simulink model "Pitoni_0"  (R2023a)
settings: Solver=VariableStepAuto  StartTime=0.0  StopTime=10  RelTol=1e-3
(part 1 of 2)
settings Model: Creator=Stefano  LastModifiedBy=hp
settings SolverCC: AlgebraicLoopSolver=TrustRegion
settings DebuggingCC: UnconnectedInputMsg=warning  UnconnectedOutputMsg=warning  UnconnectedLineMsg=warning
settings ModelReferenceCC: EnableRefExpFcnMdlSchedulingChecks=on
settings SFSimCC: CustomCodeUndefinedFunction=UseInterfaceOnly
settings RTWCC: DLArmComputeVersion=19.05

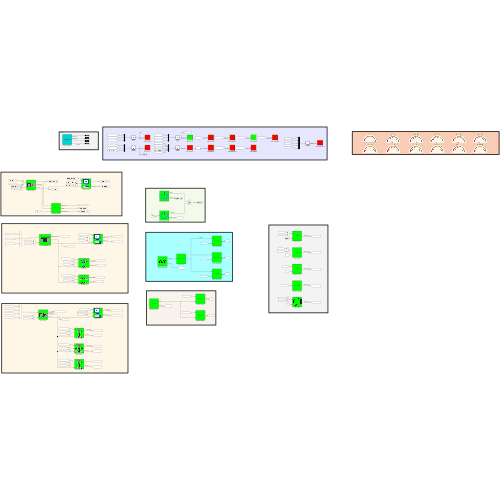
[thumbnail: Simulink's stored preview of the top-level diagram]
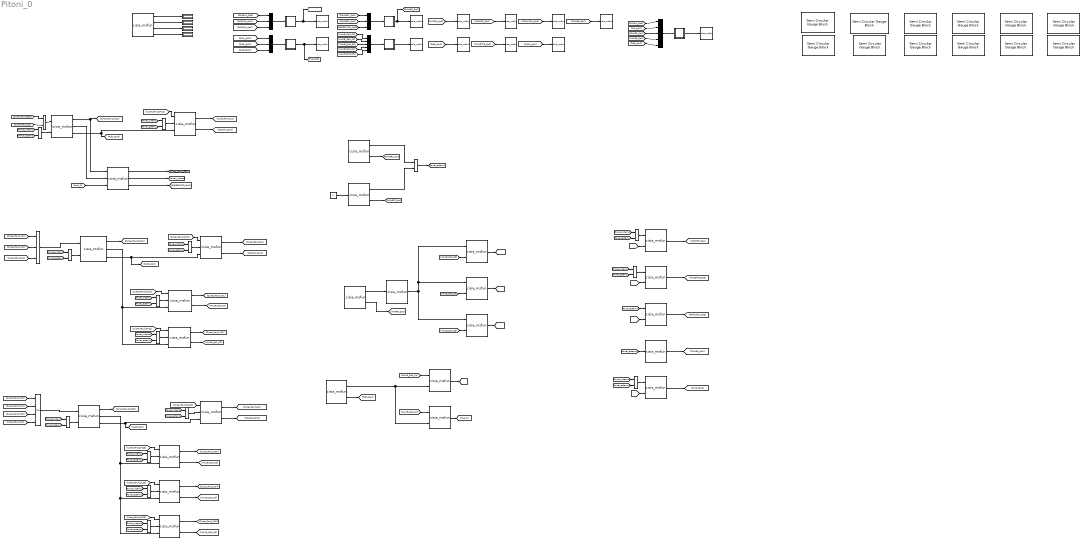
== system Pitoni_0 ==
  note: MASTER
  CISIA_MASTER (0) : M-S-Function  FunctionName=cisia_msfun  Parameters=Parameter1, Parameter2, Parameter3, resources, Parameter4, Parameter5, Parameter6, Parameter7, Parameter8, Parameter9,Parameter11  mask(S-function:msfcn_unit_delay){Parameter1='CISIA_MASTER', Parameter2=1, Parameter3='SistemiIoT', resources=off, Parameter4=on, Parameter5=off, Parameter6=off, Parameter7=off, Parameter8=0.001, Parameter9=off, Parameter11=on}
      mask prompts: Parameter1 "entity name"; Parameter2 "sampling time"; Parameter3 "project"; resources "Save status at each major hit"; Parameter4 "Show Operative Levels with colors"; Parameter5 "Load Entities from file"; Parameter6 "Load Start from Mask"; Parameter7 "Real Time"; Parameter8 "Real Time Hit (sec)"; Parameter9 "Skip saving"; Parameter11 "Show unconnected"
      mask help: This is a level-2 MATLAB file S-function which demonstrates CISIA entity
      mask Display: disp('MASTER BLOCK')
  CarWash_01 (491) : M-S-Function  FunctionName=cisia_msfun  Parameters=Parameter1, Parameter2, Parameter3, resources, Parameter10, codeupdate, step_received, step_computed, dynamic_computed, step_sended, id_entity, id_project, id_type, name_type, color  mask(S-function:msfcn_unit_delay){Parameter1='CarWash_01', Parameter2=1, Parameter3='', resources=|, Parameter10=off, codeupdate=off, step_received=|, step_computed=, dynamic_computed=, step_sended=CARWASH_QoS=Operative_Level;, id_entity=491, id_project=6, id_type=114, name_type=CarWash, color=#FFFFFF}
      mask resources=|
      | *** INPUT RESOURCES ***
      | NUM_INPUTS 2
      | POWER1 (1)
      | WATER1 (1)
      |
      | *** STATE VARIABLES ***
      | NUM_VARIABLES 3
      | Operative_Level(NUMERIC)(1)(1)
      | Power_Fault(NUMERIC)(1)(0)
      | Water_Fault(NUMERIC)(1)(0)
      |
      | *** OUTPUT RESOURCES ***
      | NUM_OUTPUTS 1
      | CARWASH_QoS (1)
      mask step_received=|
      | Power_Fault=1-POWER1;
      | Water_Fault=1-WATER1;
      |
      | Operative_Level=min(1-Power_Fault,1-Water_Fault);
      mask prompts: Parameter1 "entity name"; Parameter2 "sampling time"; Parameter3 "project"; resources "input resources and state variables"; Parameter10 "Bring state variables to output"; codeupdate "update code from mask"
      mask help: This is a level-2 MATLAB file S-function which demonstrates CISIA entity
      mask DialogControl Container1 Prompt: All parameters
      mask Display: disp('CarWash');port_label('input',1,'\color{yellow}\spadesuit','texmode','on');port_label('input',2,'\color{yellow}\spadesuit','texmode','on')
  Constant2 : Constant
  Display{18..21} (4 alike) : Display
  Fuel_Tank_01 (494) : M-S-Function  FunctionName=cisia_msfun  Parameters=Parameter1, Parameter2, Parameter3, resources, Parameter10, codeupdate, step_received, step_computed, dynamic_computed, step_sended, id_entity, id_project, id_type, name_type, color  mask(S-function:msfcn_unit_delay){Parameter1='Fuel_Tank_01', Parameter2=1, Parameter3='', resources=|, Parameter10=off, codeupdate=off, step_received=Operative_Level = 1-Mechanical_Fault, step_computed=, dynamic_computed=, step_sended=FUEL=Operative_Level;, id_entity=494, id_project=6, id_type=116, name_type=Fuel_Tank, color=#FFFFFF}
      mask resources=|
      | *** INPUT RESOURCES ***
      | NUM_INPUTS 0
      |
      | *** STATE VARIABLES ***
      | NUM_VARIABLES 2
      | Operative_Level(NUMERIC)(1)(1)
      | Mechanical_Fault(NUMERIC)(1)(0)
      |
      | *** OUTPUT RESOURCES ***
      | NUM_OUTPUTS 2
      | FUEL (1)
      | FUEL_QoS (1)
      mask prompts: Parameter1 "entity name"; Parameter2 "sampling time"; Parameter3 "project"; resources "input resources and state variables"; Parameter10 "Bring state variables to output"; codeupdate "update code from mask"
      mask help: This is a level-2 MATLAB file S-function which demonstrates CISIA entity
      mask DialogControl Container1 Prompt: All parameters
      mask Display: disp('Fuel_Tank')
  Fuel_pipe_01 (492) : M-S-Function  FunctionName=cisia_msfun  Parameters=Parameter1, Parameter2, Parameter3, resources, Parameter10, codeupdate, step_received, step_computed, dynamic_computed, step_sended, id_entity, id_project, id_type, name_type, color  mask(S-function:msfcn_unit_delay){Parameter1='Fuel_pipe_01', Parameter2=1, Parameter3='', resources=|, Parameter10=off, codeupdate=off, step_received=|, step_computed=, dynamic_computed=, step_sended=FUEL=1-Fuel_Fault;, id_entity=492, id_project=6, id_type=115, name_type=Fuel_Pipe, color=#FFFFFF}
      mask resources=|
      | *** INPUT RESOURCES ***
      | NUM_INPUTS 2
      | VALVE_QoS (1)
      | FUEL (1)
      |
      | *** STATE VARIABLES ***
      | NUM_VARIABLES 3
      | Operative_Level(NUMERIC)(1)(1)
      | Mechanical_Fault(NUMERIC)(1)(0)
      | Fuel_Fault(NUMERIC)(1)(0)
      |
      | *** OUTPUT RESOURCES ***
      | NUM_OUTPUTS 1
      | FUEL (1)
      mask step_received=|
      | Fuel_Fault=max([1-FUEL Mechanical_Fault 1-VALVE_QoS]);
      |
      | Operative_Level=1-Mechanical_Fault;
      mask prompts: Parameter1 "entity name"; Parameter2 "sampling time"; Parameter3 "project"; resources "input resources and state variables"; Parameter10 "Bring state variables to output"; codeupdate "update code from mask"
      mask help: This is a level-2 MATLAB file S-function which demonstrates CISIA entity
      mask DialogControl Container1 Prompt: All parameters
      mask Display: disp('Fuel_Pipe');port_label('input',1,'\color{yellow}\spadesuit','texmode','on')
  Fuel_pipe_02 (493) : M-S-Function  FunctionName=cisia_msfun  Parameters=Parameter1, Parameter2, Parameter3, resources, Parameter10, codeupdate, step_received, step_computed, dynamic_computed, step_sended, id_entity, id_project, id_type, name_type, color  mask(S-function:msfcn_unit_delay){Parameter1='Fuel_pipe_02', Parameter2=1, Parameter3='', resources=|, Parameter10=off, codeupdate=off, step_received=|, step_computed=, dynamic_computed=, step_sended=FUEL=1-Fuel_Fault;, id_entity=493, id_project=6, id_type=115, name_type=Fuel_Pipe, color=#FFFFFF}
      mask resources=|
      | *** INPUT RESOURCES ***
      | NUM_INPUTS 2
      | VALVE_QoS (1)
      | FUEL (1)
      |
      | *** STATE VARIABLES ***
      | NUM_VARIABLES 3
      | Operative_Level(NUMERIC)(1)(1)
      | Mechanical_Fault(NUMERIC)(1)(0)
      | Fuel_Fault(NUMERIC)(1)(0)
      |
      | *** OUTPUT RESOURCES ***
      | NUM_OUTPUTS 1
      | FUEL (1)
      mask step_received=|
      | Fuel_Fault=max([1-FUEL Mechanical_Fault 1-VALVE_QoS]);
      |
      | Operative_Level=1-Mechanical_Fault;
      mask prompts: Parameter1 "entity name"; Parameter2 "sampling time"; Parameter3 "project"; resources "input resources and state variables"; Parameter10 "Bring state variables to output"; codeupdate "update code from mask"
      mask help: This is a level-2 MATLAB file S-function which demonstrates CISIA entity
      mask DialogControl Container1 Prompt: All parameters
      mask Display: disp('Fuel_Pipe');port_label('input',1,'\color{yellow}\spadesuit','texmode','on')
  Generator_01 (495) : M-S-Function  FunctionName=cisia_msfun  Parameters=Parameter1, Parameter2, Parameter3, resources, Parameter10, codeupdate, step_received, step_computed, dynamic_computed, step_sended, id_entity, id_project, id_type, name_type, color  mask(S-function:msfcn_unit_delay){Parameter1='Generator_01', Parameter2=1, Parameter3='', resources=|, Parameter10=off, codeupdate=off, step_received=|, step_computed=, dynamic_computed=, step_sended=|, id_entity=495, id_project=6, id_type=117, name_type=Generator, color=#FFFFFF}
      mask resources=|
      | *** INPUT RESOURCES ***
      | NUM_INPUTS 3
      | CYBER_FAULT (10)
      | TELECONTROL (1)
      | FUEL (1)
      |
      | *** STATE VARIABLES ***
      | NUM_VARIABLES 14
      | Operative_Level(NUMERIC)(1)(1)
      | Dos_attack(NUMERIC)(1)(0)
      | MITM_attack(NUMERIC)(1)(0)
      | Virus_Attack(NUMERIC)(1)(0)
      | Port_Scan_Attack(NUMERIC)(1)(0)
      | Cyber_Fault(NUMERIC_ARRAY)(10)(0  0  0  0  0  0  0  0  0  0)
      | BGP_hijacking(NUMERIC)(1)(0)
      | Mechanical_Fault(NUMERIC)(1)(0)
      | BotNet_Attack(NUMERIC)(1)(0)
      | Data_Corruption(NUMERIC)(1)(0)
      | SW_Change(NUMERIC)(1)(0)
      | Config_Change(NUMERIC)(1)(0)
      | Port_Saturation(NUMERIC)(1)(0)
      | Control_Fault(NUMERIC)(1)(0)
      |
      | *** OUTPUT RESOURCES ***
      | NUM_OUTPUTS 3
      | CYBER_FAULT (10)
      | POWER1 (1)
      | GENERATOR_QoS (1)
      mask step_received=|
      | Cyber_Fault=max(CYBER_FAULT, transpose([Dos_attack MITM_attack Virus_Attack Port_Scan_Attack  BGP_hijacking BotNet_Attack Data_Corruption SW_Change Config_Change Port_Saturation]));
      |
      | Control_Fault=max([1-TELECONTROL Mechanical_Fault Dos_attack min(0.5,max(Cyber_Fault))]);
      |
      | Operative_Level=min([1-max(Cyber_Fault) 1-Mechanical_Fault FUEL]);
      mask step_sended=|
      | POWER1 = Operative_Level
      | GENERATOR_QoS = Operative_Level
      | CYBER_FAULT=Cyber_Fault.*transpose([0 0 0.5 0.2 0 0 0 0 0 0]);
      mask prompts: Parameter1 "entity name"; Parameter2 "sampling time"; Parameter3 "project"; resources "input resources and state variables"; Parameter10 "Bring state variables to output"; codeupdate "update code from mask"
      mask help: This is a level-2 MATLAB file S-function which demonstrates CISIA entity
      mask DialogControl Container1 Prompt: All parameters
      mask Display: disp('Generator');port_label('input',3,'\color{yellow}\spadesuit','texmode','on')
  Half Gauge{1..12} (12 alike) : SemiCircularGaugeBlock  ScaleMax=1
  Market_01 (517) : M-S-Function  FunctionName=cisia_msfun  Parameters=Parameter1, Parameter2, Parameter3, resources, Parameter10, codeupdate, step_received, step_computed, dynamic_computed, step_sended, id_entity, id_project, id_type, name_type, color  mask(S-function:msfcn_unit_delay){Parameter1='Market_01', Parameter2=1, Parameter3='', resources=|, Parameter10=off, codeupdate=off, step_received=|, step_computed=, dynamic_computed=, step_sended=MARKET_QoS=Operative_Level;, id_entity=517, id_project=6, id_type=128, name_type=Market, color=#FFFFFF}
      mask resources=|
      | *** INPUT RESOURCES ***
      | NUM_INPUTS 2
      | POWER1 (1)
      | WATER1 (1)
      |
      | *** STATE VARIABLES ***
      | NUM_VARIABLES 3
      | Operative_Level(NUMERIC)(1)(1)
      | Power_Fault(NUMERIC)(1)(0)
      | Water_Fault(NUMERIC)(1)(0)
      |
      | *** OUTPUT RESOURCES ***
      | NUM_OUTPUTS 1
      | MARKET_QoS (1)
      mask step_received=|
      | Power_Fault=1-POWER1;
      | Water_Fault=1-WATER1;
      |
      | Operative_Level=min(1-Power_Fault,1-Water_Fault);
      mask prompts: Parameter1 "entity name"; Parameter2 "sampling time"; Parameter3 "project"; resources "input resources and state variables"; Parameter10 "Bring state variables to output"; codeupdate "update code from mask"
      mask help: This is a level-2 MATLAB file S-function which demonstrates CISIA entity
      mask DialogControl Container1 Prompt: All parameters
      mask Display: disp('Market');port_label('input',1,'\color{yellow}\spadesuit','texmode','on');port_label('input',2,'\color{yellow}\spadesuit','texmode','on')
  MinMax : MinMax  Function=max  Inputs=4
  MinMax1 : MinMax  Function=max  Inputs=3
  MinMax{2..17} (16 alike) : MinMax  Function=max  Inputs=2
  Mux : Mux  Inputs=3
  Mux1 : Mux  Inputs=3
  Mux2 : Mux  Inputs=3
  Mux4 : Mux  Inputs=5
  Mux6 : Mux  Inputs=5
  PLC_01 (501) : M-S-Function  FunctionName=cisia_msfun  Parameters=Parameter1, Parameter2, Parameter3, resources, Parameter10, codeupdate, step_received, step_computed, dynamic_computed, step_sended, id_entity, id_project, id_type, name_type, color  mask(S-function:msfcn_unit_delay){Parameter1='PLC_01', Parameter2=1, Parameter3='', resources=|, Parameter10=off, codeupdate=off, step_received=|, step_computed=, dynamic_computed=, step_sended=|, id_entity=501, id_project=6, id_type=123, name_type=PLC, color=#FFFFFF}
      mask resources=|
      | *** INPUT RESOURCES ***
      | NUM_INPUTS 2
      | CYBER_FAULT (10)
      | POWER1 (1)
      |
      | *** STATE VARIABLES ***
      | NUM_VARIABLES 14
      | Operative_Level(NUMERIC)(1)(1)
      | Dos_attack(NUMERIC)(1)(0)
      | MITM_attack(NUMERIC)(1)(0)
      | Virus_Attack(NUMERIC)(1)(0)
      | Port_Scan_Attack(NUMERIC)(1)(0)
      | Cyber_Fault(NUMERIC_ARRAY)(10)(0  0  0  0  0  0  0  0  0  0)
      | BGP_hijacking(NUMERIC)(1)(0)
      | Mechanical_Fault(NUMERIC)(1)(0)
      | BotNet_Attack(NUMERIC)(1)(0)
      | Data_Corruption(NUMERIC)(1)(0)
      | SW_Change(NUMERIC)(1)(0)
      | Config_Change(NUMERIC)(1)(0)
      | Port_Saturation(NUMERIC)(1)(0)
      | Control_Fault(NUMERIC)(1)(0)
      |
      | *** OUTPUT RESOURCES ***
      | NUM_OUTPUTS 3
      | CYBER_FAULT (10)
      | TELECONTROL (1)
      | PLC_QoS (1)
      mask step_received=|
      | Cyber_Fault=max(CYBER_FAULT, transpose([Dos_attack MITM_attack Virus_Attack Port_Scan_Attack  BGP_hijacking BotNet_Attack Data_Corruption SW_Change Config_Change Port_Saturation]));
      |
      |
      | Control_Fault=max([Mechanical_Fault 1-POWER1 Dos_attack min(0.5,max(Cyber_Fault))]);
      |
      |
      |
      | Operative_Level=min([1-max(Cyber_Fault) 1-Mechanical_Fault 1-Control_Fault]);
      mask step_sended=|
      | CYBER_FAULT=Cyber_Fault.*transpose([0 0 0.5 0.2 0 0 0 0 0 0]);
      |
      | TELECONTROL=1-Control_Fault;
      | PLC_QoS=Operative_Level;
      mask prompts: Parameter1 "entity name"; Parameter2 "sampling time"; Parameter3 "project"; resources "input resources and state variables"; Parameter10 "Bring state variables to output"; codeupdate "update code from mask"
      mask help: This is a level-2 MATLAB file S-function which demonstrates CISIA entity
      mask DialogControl Container1 Prompt: All parameters
      mask Display: image('Icons/PLC.png');port_label('input',1,'\color{yellow}\spadesuit','texmode','on');port_label('input',2,'\color{yellow}\spadesuit','texmode','on')
  PLC_02 (506) : M-S-Function  FunctionName=cisia_msfun  Parameters=Parameter1, Parameter2, Parameter3, resources, Parameter10, codeupdate, step_received, step_computed, dynamic_computed, step_sended, id_entity, id_project, id_type, name_type, color  mask(S-function:msfcn_unit_delay){Parameter1='PLC_02', Parameter2=1, Parameter3='', resources=|, Parameter10=off, codeupdate=off, step_received=|, step_computed=, dynamic_computed=, step_sended=|, id_entity=506, id_project=6, id_type=123, name_type=PLC, color=#FFFFFF}
      mask resources=|
      | *** INPUT RESOURCES ***
      | NUM_INPUTS 2
      | CYBER_FAULT (10)
      | POWER1 (1)
      |
      | *** STATE VARIABLES ***
      | NUM_VARIABLES 14
      | Operative_Level(NUMERIC)(1)(1)
      | Dos_attack(NUMERIC)(1)(0)
      | MITM_attack(NUMERIC)(1)(0)
      | Virus_Attack(NUMERIC)(1)(0)
      | Port_Scan_Attack(NUMERIC)(1)(0)
      | Cyber_Fault(NUMERIC_ARRAY)(10)(0  0  0  0  0  0  0  0  0  0)
      | BGP_hijacking(NUMERIC)(1)(0)
      | Mechanical_Fault(NUMERIC)(1)(0)
      | BotNet_Attack(NUMERIC)(1)(0)
      | Data_Corruption(NUMERIC)(1)(0)
      | SW_Change(NUMERIC)(1)(0)
      | Config_Change(NUMERIC)(1)(0)
      | Port_Saturation(NUMERIC)(1)(0)
      | Control_Fault(NUMERIC)(1)(0)
      |
      | *** OUTPUT RESOURCES ***
      | NUM_OUTPUTS 3
      | CYBER_FAULT (10)
      | TELECONTROL (1)
      | PLC_QoS (1)
      mask step_received=|
      | Cyber_Fault=max(CYBER_FAULT, transpose([Dos_attack MITM_attack Virus_Attack Port_Scan_Attack  BGP_hijacking BotNet_Attack Data_Corruption SW_Change Config_Change Port_Saturation]));
      |
      |
      | Control_Fault=max([Mechanical_Fault 1-POWER1 Dos_attack min(0.5,max(Cyber_Fault))]);
      |
      |
      |
      | Operative_Level=min([1-max(Cyber_Fault) 1-Mechanical_Fault 1-Control_Fault]);
      mask step_sended=|
      | CYBER_FAULT=Cyber_Fault.*transpose([0 0 0.5 0.2 0 0 0 0 0 0]);
      |
      | TELECONTROL=1-Control_Fault;
      | PLC_QoS=Operative_Level;
      mask prompts: Parameter1 "entity name"; Parameter2 "sampling time"; Parameter3 "project"; resources "input resources and state variables"; Parameter10 "Bring state variables to output"; codeupdate "update code from mask"
      mask help: This is a level-2 MATLAB file S-function which demonstrates CISIA entity
      mask DialogControl Container1 Prompt: All parameters
      mask Display: image('Icons/PLC.png');port_label('input',1,'\color{yellow}\spadesuit','texmode','on');port_label('input',2,'\color{yellow}\spadesuit','texmode','on')
  PLC_03 (507) : M-S-Function  FunctionName=cisia_msfun  Parameters=Parameter1, Parameter2, Parameter3, resources, Parameter10, codeupdate, step_received, step_computed, dynamic_computed, step_sended, id_entity, id_project, id_type, name_type, color  mask(S-function:msfcn_unit_delay){Parameter1='PLC_03', Parameter2=1, Parameter3='', resources=|, Parameter10=off, codeupdate=off, step_received=|, step_computed=, dynamic_computed=, step_sended=|, id_entity=507, id_project=6, id_type=123, name_type=PLC, color=#FFFFFF}
      mask resources=|
      | *** INPUT RESOURCES ***
      | NUM_INPUTS 2
      | CYBER_FAULT (10)
      | POWER1 (1)
      |
      | *** STATE VARIABLES ***
      | NUM_VARIABLES 14
      | Operative_Level(NUMERIC)(1)(1)
      | Dos_attack(NUMERIC)(1)(0)
      | MITM_attack(NUMERIC)(1)(0)
      | Virus_Attack(NUMERIC)(1)(0)
      | Port_Scan_Attack(NUMERIC)(1)(0)
      | Cyber_Fault(NUMERIC_ARRAY)(10)(0  0  0  0  0  0  0  0  0  0)
      | BGP_hijacking(NUMERIC)(1)(0)
      | Mechanical_Fault(NUMERIC)(1)(0)
      | BotNet_Attack(NUMERIC)(1)(0)
      | Data_Corruption(NUMERIC)(1)(0)
      | SW_Change(NUMERIC)(1)(0)
      | Config_Change(NUMERIC)(1)(0)
      | Port_Saturation(NUMERIC)(1)(0)
      | Control_Fault(NUMERIC)(1)(0)
      |
      | *** OUTPUT RESOURCES ***
      | NUM_OUTPUTS 3
      | CYBER_FAULT (10)
      | TELECONTROL (1)
      | PLC_QoS (1)
      mask step_received=|
      | Cyber_Fault=max(CYBER_FAULT, transpose([Dos_attack MITM_attack Virus_Attack Port_Scan_Attack  BGP_hijacking BotNet_Attack Data_Corruption SW_Change Config_Change Port_Saturation]));
      |
      |
      | Control_Fault=max([Mechanical_Fault 1-POWER1 Dos_attack min(0.5,max(Cyber_Fault))]);
      |
      |
      |
      | Operative_Level=min([1-max(Cyber_Fault) 1-Mechanical_Fault 1-Control_Fault]);
      mask step_sended=|
      | CYBER_FAULT=Cyber_Fault.*transpose([0 0 0.5 0.2 0 0 0 0 0 0]);
      |
      | TELECONTROL=1-Control_Fault;
      | PLC_QoS=Operative_Level;
      mask prompts: Parameter1 "entity name"; Parameter2 "sampling time"; Parameter3 "project"; resources "input resources and state variables"; Parameter10 "Bring state variables to output"; codeupdate "update code from mask"
      mask help: This is a level-2 MATLAB file S-function which demonstrates CISIA entity
      mask DialogControl Container1 Prompt: All parameters
      mask Display: image('Icons/PLC.png');port_label('input',1,'\color{yellow}\spadesuit','texmode','on');port_label('input',2,'\color{yellow}\spadesuit','texmode','on')
  PowerTower_01 (497) : M-S-Function  FunctionName=cisia_msfun  Parameters=Parameter1, Parameter2, Parameter3, resources, Parameter10, codeupdate, step_received, step_computed, dynamic_computed, step_sended, id_entity, id_project, id_type, name_type, color  mask(S-function:msfcn_unit_delay){Parameter1='PowerTower_01', Parameter2=1, Parameter3='', resources=|, Parameter10=off, codeupdate=off, step_received=|, step_computed=, dynamic_computed=, step_sended=TOWER_QoS=Operative_Level;, id_entity=497, id_project=6, id_type=119, name_type=PowerTower, color=#FFFFFF}
      mask resources=|
      | *** INPUT RESOURCES ***
      | NUM_INPUTS 1
      | POWER1 (1)
      |
      | *** STATE VARIABLES ***
      | NUM_VARIABLES 3
      | Operative_Level(NUMERIC)(1)(1)
      | Mechanical_Fault(NUMERIC)(1)(0)
      | Power_Fault(NUMERIC)(1)(0)
      |
      | *** OUTPUT RESOURCES ***
      | NUM_OUTPUTS 1
      | TOWER_QoS (1)
      mask step_received=|
      | Power_Fault=1-POWER;
      |
      | Operative_Level=min(1-Mechanical_Fault 1-Power_Fault);
      mask prompts: Parameter1 "entity name"; Parameter2 "sampling time"; Parameter3 "project"; resources "input resources and state variables"; Parameter10 "Bring state variables to output"; codeupdate "update code from mask"
      mask help: This is a level-2 MATLAB file S-function which demonstrates CISIA entity
      mask DialogControl Container1 Prompt: All parameters
      mask Display: disp('PowerTower');port_label('input',1,'\color{yellow}\spadesuit','texmode','on')
  Power_availability (362) : M-S-Function  FunctionName=cisia_msfun  Parameters=Parameter1, Parameter2, Parameter3, resources, Parameter10, codeupdate, step_received, step_computed, dynamic_computed, step_sended, id_entity, id_project, id_type, name_type, color  mask(S-function:msfcn_unit_delay){Parameter1='Power_availability', Parameter2=1, Parameter3='SistemiIoT', resources=|, Parameter10=off, codeupdate=off, step_received=|, step_computed=, dynamic_computed=, step_sended=|, id_entity=362, id_project=6, id_type=94, name_type=PowerAvailability, color=#FFFFFF}
      mask resources=|
      | *** INPUT RESOURCES ***
      | NUM_INPUTS 1
      | POWER1 (1)
      |
      | *** STATE VARIABLES ***
      | NUM_VARIABLES 2
      | Operative_Level(NUMERIC)(1)(1)
      | Power_Fault(NUMERIC)(1)(0)
      |
      | *** OUTPUT RESOURCES ***
      | NUM_OUTPUTS 2
      | POWER1 (1)
      | POWER_QoS (1)
      mask step_received=|
      | Power_Fault=1-POWER1;
      | Operative_Level=1-Power_Fault;
      mask step_sended=|
      | POWER1=1-Power_Fault;
      | POWER_QoS=1-Power_Fault;
      mask prompts: Parameter1 "entity name"; Parameter2 "sampling time"; Parameter3 "project"; resources "input resources and state variables"; Parameter10 "Bring state variables to output"; codeupdate "update code from mask"
      mask help: This is a level-2 MATLAB file S-function which demonstrates CISIA entity
      mask DialogControl Container1 Prompt: All parameters
      mask Display: image('Icons/PowerAvailability.png');port_label('input',1,'\color{yellow}\spadesuit','texmode','on')
  Pump_01 (502) : M-S-Function  FunctionName=cisia_msfun  Parameters=Parameter1, Parameter2, Parameter3, resources, Parameter10, codeupdate, step_received, step_computed, dynamic_computed, step_sended, id_entity, id_project, id_type, name_type, color  mask(S-function:msfcn_unit_delay){Parameter1='Pump_01', Parameter2=1, Parameter3='', resources=|, Parameter10=off, codeupdate=off, step_received=|, step_computed=, dynamic_computed=, step_sended=|, id_entity=502, id_project=6, id_type=124, name_type=Pump, color=#FFFFFF}
      mask resources=|
      | *** INPUT RESOURCES ***
      | NUM_INPUTS 2
      | POWER1 (1)
      | FUEL (1)
      |
      | *** STATE VARIABLES ***
      | NUM_VARIABLES 14
      | Operative_Level(NUMERIC)(1)(1)
      | Dos_attack(NUMERIC)(1)(0)
      | MITM_attack(NUMERIC)(1)(0)
      | Virus_Attack(NUMERIC)(1)(0)
      | Port_Scan_Attack(NUMERIC)(1)(0)
      | Cyber_Fault(NUMERIC_ARRAY)(10)(0  0  0  0  0  0  0  0  0  0)
      | BGP_hijacking(NUMERIC)(1)(0)
      | Mechanical_Fault(NUMERIC)(1)(0)
      | BotNet_Attack(NUMERIC)(1)(0)
      | Data_Corruption(NUMERIC)(1)(0)
      | SW_Change(NUMERIC)(1)(0)
      | Config_Change(NUMERIC)(1)(0)
      | Port_Saturation(NUMERIC)(1)(0)
      | Control_Fault(NUMERIC)(1)(0)
      |
      | *** OUTPUT RESOURCES ***
      | NUM_OUTPUTS 1
      | PUMP_QoS (1)
      mask step_received=|
      | Cyber_Fault=max(CYBER_FAULT, transpose([Dos_attack MITM_attack Virus_Attack Port_Scan_Attack  BGP_hijacking BotNet_Attack Data_Corruption SW_Change Config_Change Port_Saturation]));
      |
      |
      | Control_Fault=max([1-TELECONTROL Mechanical_Fault Dos_attack min(0.5,max(Cyber_Fault))]);
      |
      |
      |
      | Operative_Level=min([1-max(Cyber_Fault) 1-Mechanical_Fault POWER]);
      mask step_sended=|
      | PUMP_QoS=1-Control_Fault;
      | CYBER_FAULT=Cyber_Fault.*transpose([0 0 0.5 0.2 0 0 0 0 0 0]);
      mask prompts: Parameter1 "entity name"; Parameter2 "sampling time"; Parameter3 "project"; resources "input resources and state variables"; Parameter10 "Bring state variables to output"; codeupdate "update code from mask"
      mask help: This is a level-2 MATLAB file S-function which demonstrates CISIA entity
      mask DialogControl Container1 Prompt: All parameters
      mask Display: image('Icons/Pump.png');port_label('input',1,'\color{yellow}\spadesuit','texmode','on');port_label('input',2,'\color{yellow}\spadesuit','texmode','on')
  SAVE_17 (17) : M-S-Function  FunctionName=cisia_msfun  Parameters=Parameter1, Parameter2, Parameter3, Parameter4,Parameter5,Parameter6,Parameter7  mask(S-function:msfcn_unit_delay){Parameter1='SAVE_17', Parameter2=1, Parameter3='SistemiIoT', Parameter4=on, Parameter5=[1], Parameter6=[1], Parameter7=off}
      mask prompts: Parameter1 "entity name"; Parameter2 "sampling time"; Parameter3 "project"; Parameter4 "display bars"; Parameter5 "values"; Parameter6 "logic"; Parameter7 "display B/W"
      mask help: This is a level-2 MATLAB file S-function which demonstrates CISIA entity
      mask DialogControl Container3 Prompt: Display
      mask Display:
      | display=get_param(gcb, 'Parameter4');
      | greymap=get_param(gcb, 'Parameter7');
      | 
      | if strcmp(display,'on')
      | 
      |     val=str2num(get_param(gcb, 'Parameter5'));
      |     logic=str2num(get_param(gcb, 'Parameter6'));
      |     n=length(val);
      | 
      |     val2=val;
      |     l=length(logic);
      |     if l>0
      |         for i=1:l
      |             if logic(i)==-1
      |                 val2(i)=1-val2(i);
      |             end
      |         end
      |     end
      | 
      | 
      | 
      | 
      |     if strcmp(greymap,'on')
      |         val_r=round(val2*50)+1;
      |         colormap=gray(60);
      |         color2=[0 0 0];
      |     else
      |         val_r=round(val2*20)+1;
      |         colormap=hsv(60);
      |         color2=[0 0 1];
      |     end
      | 
      |     patch([0 0 n n], [0 -0.2 -0.2 0], [1 1 1]);
      | 
      |     for i=1:n
      |         color=colormap(val_r(i),:);
      |         patch([i-1 i-1 i i],[0 1 1 0],color)
      |         patch([i-1 i],[val(i) val(i)],color2)
      | 
      |     end
      | 
      |     for i=1:n
      |         patch([i i], [-0.2 1], [0 0 0]);
      |         text(i-0.5, -0.1, num2str(val(i)));
      |     end
      | 
      | 
      | else
      | 
      |     disp('SAVE');
      | 
      | end
  SAVE_CAR (29) : M-S-Function  FunctionName=cisia_msfun  Parameters=Parameter1, Parameter2, Parameter3, Parameter4,Parameter5,Parameter6,Parameter7  mask(S-function:msfcn_unit_delay){Parameter1='SAVE_CAR', Parameter2=1, Parameter3='SistemiIoT', Parameter4=on, Parameter5=[1], Parameter6=[1], Parameter7=off}
      mask prompts: Parameter1 "entity name"; Parameter2 "sampling time"; Parameter3 "project"; Parameter4 "display bars"; Parameter5 "values"; Parameter6 "logic"; Parameter7 "display B/W"
      mask help: This is a level-2 MATLAB file S-function which demonstrates CISIA entity
      mask DialogControl Container3 Prompt: Display
      mask Display:
      | display=get_param(gcb, 'Parameter4');
      | greymap=get_param(gcb, 'Parameter7');
      | 
      | if strcmp(display,'on')
      | 
      |     val=str2num(get_param(gcb, 'Parameter5'));
      |     logic=str2num(get_param(gcb, 'Parameter6'));
      |     n=length(val);
      | 
      |     val2=val;
      |     l=length(logic);
      |     if l>0
      |         for i=1:l
      |             if logic(i)==-1
      |                 val2(i)=1-val2(i);
      |             end
      |         end
      |     end
      | 
      | 
      | 
      | 
      |     if strcmp(greymap,'on')
      |         val_r=round(val2*50)+1;
      |         colormap=gray(60);
      |         color2=[0 0 0];
      |     else
      |         val_r=round(val2*20)+1;
      |         colormap=hsv(60);
      |         color2=[0 0 1];
      |     end
      | 
      |     patch([0 0 n n], [0 -0.2 -0.2 0], [1 1 1]);
      | 
      |     for i=1:n
      |         color=colormap(val_r(i),:);
      |         patch([i-1 i-1 i i],[0 1 1 0],color)
      |         patch([i-1 i],[val(i) val(i)],color2)
      | 
      |     end
      | 
      |     for i=1:n
      |         patch([i i], [-0.2 1], [0 0 0]);
      |         text(i-0.5, -0.1, num2str(val(i)));
      |     end
      | 
      | 
      | else
      | 
      |     disp('SAVE');
      | 
      | end
  SAVE_FUEL (34) : M-S-Function  FunctionName=cisia_msfun  Parameters=Parameter1, Parameter2, Parameter3, Parameter4,Parameter5,Parameter6,Parameter7  mask(S-function:msfcn_unit_delay){Parameter1='SAVE_FUEL', Parameter2=1, Parameter3='SistemiIoT', Parameter4=on, Parameter5=[0], Parameter6=[1], Parameter7=off}
      mask prompts: Parameter1 "entity name"; Parameter2 "sampling time"; Parameter3 "project"; Parameter4 "display bars"; Parameter5 "values"; Parameter6 "logic"; Parameter7 "display B/W"
      mask help: This is a level-2 MATLAB file S-function which demonstrates CISIA entity
      mask DialogControl Container3 Prompt: Display
      mask Display:
      | display=get_param(gcb, 'Parameter4');
      | greymap=get_param(gcb, 'Parameter7');
      | 
      | if strcmp(display,'on')
      | 
      |     val=str2num(get_param(gcb, 'Parameter5'));
      |     logic=str2num(get_param(gcb, 'Parameter6'));
      |     n=length(val);
      | 
      |     val2=val;
      |     l=length(logic);
      |     if l>0
      |         for i=1:l
      |             if logic(i)==-1
      |                 val2(i)=1-val2(i);
      |             end
      |         end
      |     end
      | 
      | 
      | 
      | 
      |     if strcmp(greymap,'on')
      |         val_r=round(val2*50)+1;
      |         colormap=gray(60);
      |         color2=[0 0 0];
      |     else
      |         val_r=round(val2*20)+1;
      |         colormap=hsv(60);
      |         color2=[0 0 1];
      |     end
      | 
      |     patch([0 0 n n], [0 -0.2 -0.2 0], [1 1 1]);
      | 
      |     for i=1:n
      |         color=colormap(val_r(i),:);
      |         patch([i-1 i-1 i i],[0 1 1 0],color)
      |         patch([i-1 i],[val(i) val(i)],color2)
      | 
      |     end
      | 
      |     for i=1:n
      |         patch([i i], [-0.2 1], [0 0 0]);
      |         text(i-0.5, -0.1, num2str(val(i)));
      |     end
      | 
      | 
      | else
      | 
      |     disp('SAVE');
      | 
      | end
  SAVE_GENERAL (33) : M-S-Function  FunctionName=cisia_msfun  Parameters=Parameter1, Parameter2, Parameter3, Parameter4,Parameter5,Parameter6,Parameter7  mask(S-function:msfcn_unit_delay){Parameter1='SAVE_GENERAL', Parameter2=1, Parameter3='SistemiIoT', Parameter4=on, Parameter5=[0], Parameter6=[1], Parameter7=off}
      mask prompts: Parameter1 "entity name"; Parameter2 "sampling time"; Parameter3 "project"; Parameter4 "display bars"; Parameter5 "values"; Parameter6 "logic"; Parameter7 "display B/W"
      mask help: This is a level-2 MATLAB file S-function which demonstrates CISIA entity
      mask DialogControl Container3 Prompt: Display
      mask Display:
      | display=get_param(gcb, 'Parameter4');
      | greymap=get_param(gcb, 'Parameter7');
      | 
      | if strcmp(display,'on')
      | 
      |     val=str2num(get_param(gcb, 'Parameter5'));
      |     logic=str2num(get_param(gcb, 'Parameter6'));
      |     n=length(val);
      | 
      |     val2=val;
      |     l=length(logic);
      |     if l>0
      |         for i=1:l
      |             if logic(i)==-1
      |                 val2(i)=1-val2(i);
      |             end
      |         end
      |     end
      | 
      | 
      | 
      | 
      |     if strcmp(greymap,'on')
      |         val_r=round(val2*50)+1;
      |         colormap=gray(60);
      |         color2=[0 0 0];
      |     else
      |         val_r=round(val2*20)+1;
      |         colormap=hsv(60);
      |         color2=[0 0 1];
      |     end
      | 
      |     patch([0 0 n n], [0 -0.2 -0.2 0], [1 1 1]);
      | 
      |     for i=1:n
      |         color=colormap(val_r(i),:);
      |         patch([i-1 i-1 i i],[0 1 1 0],color)
      |         patch([i-1 i],[val(i) val(i)],color2)
      | 
      |     end
      | 
      |     for i=1:n
      |         patch([i i], [-0.2 1], [0 0 0]);
      |         text(i-0.5, -0.1, num2str(val(i)));
      |     end
      | 
      | 
      | else
      | 
      |     disp('SAVE');
      | 
      | end
  SAVE_MARKET (28) : M-S-Function  FunctionName=cisia_msfun  Parameters=Parameter1, Parameter2, Parameter3, Parameter4,Parameter5,Parameter6,Parameter7  mask(S-function:msfcn_unit_delay){Parameter1='SAVE_MARKET', Parameter2=1, Parameter3='SistemiIoT', Parameter4=on, Parameter5=[0], Parameter6=[1], Parameter7=off}
      mask prompts: Parameter1 "entity name"; Parameter2 "sampling time"; Parameter3 "project"; Parameter4 "display bars"; Parameter5 "values"; Parameter6 "logic"; Parameter7 "display B/W"
      mask help: This is a level-2 MATLAB file S-function which demonstrates CISIA entity
      mask DialogControl Container3 Prompt: Display
      mask Display:
      | display=get_param(gcb, 'Parameter4');
      | greymap=get_param(gcb, 'Parameter7');
      | 
      | if strcmp(display,'on')
      | 
      |     val=str2num(get_param(gcb, 'Parameter5'));
      |     logic=str2num(get_param(gcb, 'Parameter6'));
      |     n=length(val);
      | 
      |     val2=val;
      |     l=length(logic);
      |     if l>0
      |         for i=1:l
      |             if logic(i)==-1
      |                 val2(i)=1-val2(i);
      |             end
      |         end
      |     end
      | 
      | 
      | 
      | 
      |     if strcmp(greymap,'on')
      |         val_r=round(val2*50)+1;
      |         colormap=gray(60);
      |         color2=[0 0 0];
      |     else
      |         val_r=round(val2*20)+1;
      |         colormap=hsv(60);
      |         color2=[0 0 1];
      |     end
      | 
      |     patch([0 0 n n], [0 -0.2 -0.2 0], [1 1 1]);
      | 
      |     for i=1:n
      |         color=colormap(val_r(i),:);
      |         patch([i-1 i-1 i i],[0 1 1 0],color)
      |         patch([i-1 i],[val(i) val(i)],color2)
      | 
      |     end
      | 
      |     for i=1:n
      |         patch([i i], [-0.2 1], [0 0 0]);
      |         text(i-0.5, -0.1, num2str(val(i)));
      |     end
      | 
      | 
      | else
      | 
      |     disp('SAVE');
      | 
      | end
  SAVE_PLC (31) : M-S-Function  FunctionName=cisia_msfun  Parameters=Parameter1, Parameter2, Parameter3, Parameter4,Parameter5,Parameter6,Parameter7  mask(S-function:msfcn_unit_delay){Parameter1='SAVE_PLC', Parameter2=1, Parameter3='SistemiIoT', Parameter4=on, Parameter5=[0], Parameter6=[1], Parameter7=off}
      mask prompts: Parameter1 "entity name"; Parameter2 "sampling time"; Parameter3 "project"; Parameter4 "display bars"; Parameter5 "values"; Parameter6 "logic"; Parameter7 "display B/W"
      mask help: This is a level-2 MATLAB file S-function which demonstrates CISIA entity
      mask DialogControl Container3 Prompt: Display
      mask Display:
      | display=get_param(gcb, 'Parameter4');
      | greymap=get_param(gcb, 'Parameter7');
      | 
      | if strcmp(display,'on')
      | 
      |     val=str2num(get_param(gcb, 'Parameter5'));
      |     logic=str2num(get_param(gcb, 'Parameter6'));
      |     n=length(val);
      | 
      |     val2=val;
      |     l=length(logic);
      |     if l>0
      |         for i=1:l
      |             if logic(i)==-1
      |                 val2(i)=1-val2(i);
      |             end
      |         end
      |     end
      | 
      | 
      | 
      | 
      |     if strcmp(greymap,'on')
      |         val_r=round(val2*50)+1;
      |         colormap=gray(60);
      |         color2=[0 0 0];
      |     else
      |         val_r=round(val2*20)+1;
      |         colormap=hsv(60);
      |         color2=[0 0 1];
      |     end
      | 
      |     patch([0 0 n n], [0 -0.2 -0.2 0], [1 1 1]);
      | 
      |     for i=1:n
      |         color=colormap(val_r(i),:);
      |         patch([i-1 i-1 i i],[0 1 1 0],color)
      |         patch([i-1 i],[val(i) val(i)],color2)
      | 
      |     end
      | 
      |     for i=1:n
      |         patch([i i], [-0.2 1], [0 0 0]);
      |         text(i-0.5, -0.1, num2str(val(i)));
      |     end
      | 
      | 
      | else
      | 
      |     disp('SAVE');
      | 
      | end
  SAVE_PUMP (30) : M-S-Function  FunctionName=cisia_msfun  Parameters=Parameter1, Parameter2, Parameter3, Parameter4,Parameter5,Parameter6,Parameter7  mask(S-function:msfcn_unit_delay){Parameter1='SAVE_PUMP', Parameter2=1, Parameter3='SistemiIoT', Parameter4=on, Parameter5=[0], Parameter6=[1], Parameter7=off}
      mask prompts: Parameter1 "entity name"; Parameter2 "sampling time"; Parameter3 "project"; Parameter4 "display bars"; Parameter5 "values"; Parameter6 "logic"; Parameter7 "display B/W"
      mask help: This is a level-2 MATLAB file S-function which demonstrates CISIA entity
      mask DialogControl Container3 Prompt: Display
      mask Display:
      | display=get_param(gcb, 'Parameter4');
      | greymap=get_param(gcb, 'Parameter7');
      | 
      | if strcmp(display,'on')
      | 
      |     val=str2num(get_param(gcb, 'Parameter5'));
      |     logic=str2num(get_param(gcb, 'Parameter6'));
      |     n=length(val);
      | 
      |     val2=val;
      |     l=length(logic);
      |     if l>0
      |         for i=1:l
      |             if logic(i)==-1
      |                 val2(i)=1-val2(i);
      |             end
      |         end
      |     end
      | 
      | 
      | 
      | 
      |     if strcmp(greymap,'on')
      |         val_r=round(val2*50)+1;
      |         colormap=gray(60);
      |         color2=[0 0 0];
      |     else
      |         val_r=round(val2*20)+1;
      |         colormap=hsv(60);
      |         color2=[0 0 1];
      |     end
      | 
      |     patch([0 0 n n], [0 -0.2 -0.2 0], [1 1 1]);
      | 
      |     for i=1:n
      |         color=colormap(val_r(i),:);
      |         patch([i-1 i-1 i i],[0 1 1 0],color)
      |         patch([i-1 i],[val(i) val(i)],color2)
      | 
      |     end
      | 
      |     for i=1:n
      |         patch([i i], [-0.2 1], [0 0 0]);
      |         text(i-0.5, -0.1, num2str(val(i)));
      |     end
      | 
      | 
      | else
      | 
      |     disp('SAVE');
      | 
      | end
  SAVE_SCADA (26) : M-S-Function  FunctionName=cisia_msfun  Parameters=Parameter1, Parameter2, Parameter3, Parameter4,Parameter5,Parameter6,Parameter7  mask(S-function:msfcn_unit_delay){Parameter1='SAVE_SCADA', Parameter2=1, Parameter3='SistemiIoT', Parameter4=on, Parameter5=[0], Parameter6=[1], Parameter7=off}
      mask prompts: Parameter1 "entity name"; Parameter2 "sampling time"; Parameter3 "project"; Parameter4 "display bars"; Parameter5 "values"; Parameter6 "logic"; Parameter7 "display B/W"
      mask help: This is a level-2 MATLAB file S-function which demonstrates CISIA entity
      mask DialogControl Container3 Prompt: Display
      mask Display:
      | display=get_param(gcb, 'Parameter4');
      | greymap=get_param(gcb, 'Parameter7');
      | 
      | if strcmp(display,'on')
      | 
      |     val=str2num(get_param(gcb, 'Parameter5'));
      |     logic=str2num(get_param(gcb, 'Parameter6'));
      |     n=length(val);
      | 
      |     val2=val;
      |     l=length(logic);
      |     if l>0
      |         for i=1:l
      |             if logic(i)==-1
      |                 val2(i)=1-val2(i);
      |             end
      |         end
      |     end
      | 
      | 
      | 
      | 
      |     if strcmp(greymap,'on')
      |         val_r=round(val2*50)+1;
      |         colormap=gray(60);
      |         color2=[0 0 0];
      |     else
      |         val_r=round(val2*20)+1;
      |         colormap=hsv(60);
      |         color2=[0 0 1];
      |     end
      | 
      |     patch([0 0 n n], [0 -0.2 -0.2 0], [1 1 1]);
      | 
      |     for i=1:n
      |         color=colormap(val_r(i),:);
      |         patch([i-1 i-1 i i],[0 1 1 0],color)
      |         patch([i-1 i],[val(i) val(i)],color2)
      | 
      |     end
      | 
      |     for i=1:n
      |         patch([i i], [-0.2 1], [0 0 0]);
      |         text(i-0.5, -0.1, num2str(val(i)));
      |     end
      | 
      | 
      | else
      | 
      |     disp('SAVE');
      | 
      | end
  SAVE_TOILETTE (27) : M-S-Function  FunctionName=cisia_msfun  Parameters=Parameter1, Parameter2, Parameter3, Parameter4,Parameter5,Parameter6,Parameter7  mask(S-function:msfcn_unit_delay){Parameter1='SAVE_TOILETTE', Parameter2=1, Parameter3='SistemiIoT', Parameter4=on, Parameter5=[0], Parameter6=[1], Parameter7=off}
      mask prompts: Parameter1 "entity name"; Parameter2 "sampling time"; Parameter3 "project"; Parameter4 "display bars"; Parameter5 "values"; Parameter6 "logic"; Parameter7 "display B/W"
      mask help: This is a level-2 MATLAB file S-function which demonstrates CISIA entity
      mask DialogControl Container3 Prompt: Display
      mask Display:
      | display=get_param(gcb, 'Parameter4');
      | greymap=get_param(gcb, 'Parameter7');
      | 
      | if strcmp(display,'on')
      | 
      |     val=str2num(get_param(gcb, 'Parameter5'));
      |     logic=str2num(get_param(gcb, 'Parameter6'));
      |     n=length(val);
      | 
      |     val2=val;
      |     l=length(logic);
      |     if l>0
      |         for i=1:l
      |             if logic(i)==-1
      |                 val2(i)=1-val2(i);
      |             end
      |         end
      |     end
      | 
      | 
      | 
      | 
      |     if strcmp(greymap,'on')
      |         val_r=round(val2*50)+1;
      |         colormap=gray(60);
      |         color2=[0 0 0];
      |     else
      |         val_r=round(val2*20)+1;
      |         colormap=hsv(60);
      |         color2=[0 0 1];
      |     end
      | 
      |     patch([0 0 n n], [0 -0.2 -0.2 0], [1 1 1]);
      | 
      |     for i=1:n
      |         color=colormap(val_r(i),:);
      |         patch([i-1 i-1 i i],[0 1 1 0],color)
      |         patch([i-1 i],[val(i) val(i)],color2)
      | 
      |     end
      | 
      |     for i=1:n
      |         patch([i i], [-0.2 1], [0 0 0]);
      |         text(i-0.5, -0.1, num2str(val(i)));
      |     end
      | 
      | 
      | else
      | 
      |     disp('SAVE');
      | 
      | end
  SAVE_TOWER (35) : M-S-Function  FunctionName=cisia_msfun  Parameters=Parameter1, Parameter2, Parameter3, Parameter4,Parameter5,Parameter6,Parameter7  mask(S-function:msfcn_unit_delay){Parameter1='SAVE_TOWER', Parameter2=1, Parameter3='SistemiIoT', Parameter4=on, Parameter5=[0], Parameter6=[1], Parameter7=off}
      mask prompts: Parameter1 "entity name"; Parameter2 "sampling time"; Parameter3 "project"; Parameter4 "display bars"; Parameter5 "values"; Parameter6 "logic"; Parameter7 "display B/W"
      mask help: This is a level-2 MATLAB file S-function which demonstrates CISIA entity
      mask DialogControl Container3 Prompt: Display
      mask Display:
      | display=get_param(gcb, 'Parameter4');
      | greymap=get_param(gcb, 'Parameter7');
      | 
      | if strcmp(display,'on')
      | 
      |     val=str2num(get_param(gcb, 'Parameter5'));
      |     logic=str2num(get_param(gcb, 'Parameter6'));
      |     n=length(val);
      | 
      |     val2=val;
      |     l=length(logic);
      |     if l>0
      |         for i=1:l
      |             if logic(i)==-1
      |                 val2(i)=1-val2(i);
      |             end
      |         end
      |     end
      | 
      | 
      | 
      | 
      |     if strcmp(greymap,'on')
      |         val_r=round(val2*50)+1;
      |         colormap=gray(60);
      |         color2=[0 0 0];
      |     else
      |         val_r=round(val2*20)+1;
      |         colormap=hsv(60);
      |         color2=[0 0 1];
      |     end
      | 
      |     patch([0 0 n n], [0 -0.2 -0.2 0], [1 1 1]);
      | 
      |     for i=1:n
      |         color=colormap(val_r(i),:);
      |         patch([i-1 i-1 i i],[0 1 1 0],color)
      |         patch([i-1 i],[val(i) val(i)],color2)
      | 
      |     end
      | 
      |     for i=1:n
      |         patch([i i], [-0.2 1], [0 0 0]);
      |         text(i-0.5, -0.1, num2str(val(i)));
      |     end
      | 
      | 
      | else
      | 
      |     disp('SAVE');
      | 
      | end
  SAVE_VALVE (25) : M-S-Function  FunctionName=cisia_msfun  Parameters=Parameter1, Parameter2, Parameter3, Parameter4,Parameter5,Parameter6,Parameter7  mask(S-function:msfcn_unit_delay){Parameter1='SAVE_VALVE', Parameter2=1, Parameter3='SistemiIoT', Parameter4=on, Parameter5=[0], Parameter6=[1], Parameter7=off}
      mask prompts: Parameter1 "entity name"; Parameter2 "sampling time"; Parameter3 "project"; Parameter4 "display bars"; Parameter5 "values"; Parameter6 "logic"; Parameter7 "display B/W"
      mask help: This is a level-2 MATLAB file S-function which demonstrates CISIA entity
      mask DialogControl Container3 Prompt: Display
      mask Display:
      | display=get_param(gcb, 'Parameter4');
      | greymap=get_param(gcb, 'Parameter7');
      | 
      | if strcmp(display,'on')
      | 
      |     val=str2num(get_param(gcb, 'Parameter5'));
      |     logic=str2num(get_param(gcb, 'Parameter6'));
      |     n=length(val);
      | 
      |     val2=val;
      |     l=length(logic);
      |     if l>0
      |         for i=1:l
      |             if logic(i)==-1
      |                 val2(i)=1-val2(i);
      |             end
      |         end
      |     end
      | 
      | 
      | 
      | 
      |     if strcmp(greymap,'on')
      |         val_r=round(val2*50)+1;
      |         colormap=gray(60);
      |         color2=[0 0 0];
      |     else
      |         val_r=round(val2*20)+1;
      |         colormap=hsv(60);
      |         color2=[0 0 1];
      |     end
      | 
      |     patch([0 0 n n], [0 -0.2 -0.2 0], [1 1 1]);
      | 
      |     for i=1:n
      |         color=colormap(val_r(i),:);
      |         patch([i-1 i-1 i i],[0 1 1 0],color)
      |         patch([i-1 i],[val(i) val(i)],color2)
      | 
      |     end
      | 
      |     for i=1:n
      |         patch([i i], [-0.2 1], [0 0 0]);
      |         text(i-0.5, -0.1, num2str(val(i)));
      |     end
      | 
      | 
      | else
      | 
      |     disp('SAVE');
      | 
      | end
  SAVE_WATER (32) : M-S-Function  FunctionName=cisia_msfun  Parameters=Parameter1, Parameter2, Parameter3, Parameter4,Parameter5,Parameter6,Parameter7  mask(S-function:msfcn_unit_delay){Parameter1='SAVE_WATER', Parameter2=1, Parameter3='SistemiIoT', Parameter4=on, Parameter5=[0], Parameter6=[1], Parameter7=off}
      mask prompts: Parameter1 "entity name"; Parameter2 "sampling time"; Parameter3 "project"; Parameter4 "display bars"; Parameter5 "values"; Parameter6 "logic"; Parameter7 "display B/W"
      mask help: This is a level-2 MATLAB file S-function which demonstrates CISIA entity
      mask DialogControl Container3 Prompt: Display
      mask Display:
      | display=get_param(gcb, 'Parameter4');
      | greymap=get_param(gcb, 'Parameter7');
      | 
      | if strcmp(display,'on')
      | 
      |     val=str2num(get_param(gcb, 'Parameter5'));
      |     logic=str2num(get_param(gcb, 'Parameter6'));
      |     n=length(val);
      | 
      |     val2=val;
      |     l=length(logic);
      |     if l>0
      |         for i=1:l
      |             if logic(i)==-1
      |                 val2(i)=1-val2(i);
      |             end
      |         end
      |     end
      | 
      | 
      | 
      | 
      |     if strcmp(greymap,'on')
      |         val_r=round(val2*50)+1;
      |         colormap=gray(60);
      |         color2=[0 0 0];
      |     else
      |         val_r=round(val2*20)+1;
      |         colormap=hsv(60);
      |         color2=[0 0 1];
      |     end
      | 
      |     patch([0 0 n n], [0 -0.2 -0.2 0], [1 1 1]);
      | 
      |     for i=1:n
      |         color=colormap(val_r(i),:);
      |         patch([i-1 i-1 i i],[0 1 1 0],color)
      |         patch([i-1 i],[val(i) val(i)],color2)
      | 
      |     end
      | 
      |     for i=1:n
      |         patch([i i], [-0.2 1], [0 0 0]);
      |         text(i-0.5, -0.1, num2str(val(i)));
      |     end
      | 
      | 
      | else
      | 
      |     disp('SAVE');
      | 
      | end
  SCADA_01 (508) : M-S-Function  FunctionName=cisia_msfun  Parameters=Parameter1, Parameter2, Parameter3, resources, Parameter10, codeupdate, step_received, step_computed, dynamic_computed, step_sended, id_entity, id_project, id_type, name_type, color  mask(S-function:msfcn_unit_delay){Parameter1='SCADA_01', Parameter2=1, Parameter3='SistemiIoT', resources=|, Parameter10=off, codeupdate=off, step_received=|, step_computed=, dynamic_computed=, step_sended=|, id_entity=508, id_project=6, id_type=125, name_type=SCADA, color=#FFFFFF}
      mask resources=|
      | *** INPUT RESOURCES ***
      | NUM_INPUTS 3
      | CYBER_FAULT (10)
      | POWER1 (1)
      | PLC_QoS (1)
      |
      | *** STATE VARIABLES ***
      | NUM_VARIABLES 14
      | Operative_Level(NUMERIC)(1)(1)
      | Dos_attack(NUMERIC)(1)(0)
      | MITM_attack(NUMERIC)(1)(0)
      | Virus_Attack(NUMERIC)(1)(0)
      | Port_Scan_Attack(NUMERIC)(1)(0)
      | Cyber_Fault(NUMERIC_ARRAY)(10)(0  0  0  0  0  0  0  0  0  0)
      | BGP_hijacking(NUMERIC)(1)(0)
      | Mechanical_Fault(NUMERIC)(1)(0)
      | BotNet_Attack(NUMERIC)(1)(0)
      | Data_Corruption(NUMERIC)(1)(0)
      | SW_Change(NUMERIC)(1)(0)
      | Config_Change(NUMERIC)(1)(0)
      | Port_Saturation(NUMERIC)(1)(0)
      | Control_Fault(NUMERIC)(1)(0)
      |
      | *** OUTPUT RESOURCES ***
      | NUM_OUTPUTS 2
      | CYBER_FAULT (10)
      | SCADA_QoS (1)
      mask step_received=|
      | Cyber_Fault=max(CYBER_FAULT, transpose([Dos_attack MITM_attack Virus_Attack Port_Scan_Attack  BGP_hijacking BotNet_Attack Data_Corruption SW_Change Config_Change Port_Saturation]));
      |
      |
      | %Control_Fault=max([Mechanical_Fault Dos_attack min(0.5,max(Cyber_Fault))]);
      |
      |
      |
      | %Operative_Level=min([1-max(Cyber_Fault) 1-Mechanical_Fault POWER1 PLC_QoS]);
      mask step_sended=|
      | SCADA_QoS=Operative_Level;
      |
      | CYBER_FAULT=Cyber_Fault.*transpose([0 0 0.5 0.2 0 0 0 0 0 0]);
      mask prompts: Parameter1 "entity name"; Parameter2 "sampling time"; Parameter3 "project"; resources "input resources and state variables"; Parameter10 "Bring state variables to output"; codeupdate "update code from mask"
      mask help: This is a level-2 MATLAB file S-function which demonstrates CISIA entity
      mask DialogControl Container1 Prompt: All parameters
      mask Display: image('Icons/SCADA.png');port_label('input',1,'\color{yellow}\spadesuit','texmode','on');port_label('input',2,'\color{yellow}\spadesuit','texmode','on')
  SCADA_02 (509) : M-S-Function  FunctionName=cisia_msfun  Parameters=Parameter1, Parameter2, Parameter3, resources, Parameter10, codeupdate, step_received, step_computed, dynamic_computed, step_sended, id_entity, id_project, id_type, name_type, color  mask(S-function:msfcn_unit_delay){Parameter1='SCADA_02', Parameter2=1, Parameter3='SistemiIoT', resources=|, Parameter10=off, codeupdate=off, step_received=|, step_computed=, dynamic_computed=, step_sended=|, id_entity=509, id_project=6, id_type=125, name_type=SCADA, color=#FFFFFF}
      mask resources=|
      | *** INPUT RESOURCES ***
      | NUM_INPUTS 3
      | CYBER_FAULT (10)
      | POWER1 (1)
      | PLC_QoS (1)
      |
      | *** STATE VARIABLES ***
      | NUM_VARIABLES 14
      | Operative_Level(NUMERIC)(1)(1)
      | Dos_attack(NUMERIC)(1)(0)
      | MITM_attack(NUMERIC)(1)(0)
      | Virus_Attack(NUMERIC)(1)(0)
      | Port_Scan_Attack(NUMERIC)(1)(0)
      | Cyber_Fault(NUMERIC_ARRAY)(10)(0  0  0  0  0  0  0  0  0  0)
      | BGP_hijacking(NUMERIC)(1)(0)
      | Mechanical_Fault(NUMERIC)(1)(0)
      | BotNet_Attack(NUMERIC)(1)(0)
      | Data_Corruption(NUMERIC)(1)(0)
      | SW_Change(NUMERIC)(1)(0)
      | Config_Change(NUMERIC)(1)(0)
      | Port_Saturation(NUMERIC)(1)(0)
      | Control_Fault(NUMERIC)(1)(0)
      |
      | *** OUTPUT RESOURCES ***
      | NUM_OUTPUTS 2
      | CYBER_FAULT (10)
      | SCADA_QoS (1)
      mask step_received=|
      | Cyber_Fault=max(CYBER_FAULT, transpose([Dos_attack MITM_attack Virus_Attack Port_Scan_Attack  BGP_hijacking BotNet_Attack Data_Corruption SW_Change Config_Change Port_Saturation]));
      |
      |
      | %Control_Fault=max([Mechanical_Fault Dos_attack min(0.5,max(Cyber_Fault))]);
      |
      |
      |
      | %Operative_Level=min([1-max(Cyber_Fault) 1-Mechanical_Fault POWER1 PLC_QoS]);
      mask step_sended=|
      | SCADA_QoS=Operative_Level;
      |
      | CYBER_FAULT=Cyber_Fault.*transpose([0 0 0.5 0.2 0 0 0 0 0 0]);
      mask prompts: Parameter1 "entity name"; Parameter2 "sampling time"; Parameter3 "project"; resources "input resources and state variables"; Parameter10 "Bring state variables to output"; codeupdate "update code from mask"
      mask help: This is a level-2 MATLAB file S-function which demonstrates CISIA entity
      mask DialogControl Container1 Prompt: All parameters
      mask Display: image('Icons/SCADA.png');port_label('input',1,'\color{yellow}\spadesuit','texmode','on');port_label('input',2,'\color{yellow}\spadesuit','texmode','on')
  SCADA_03 (510) : M-S-Function  FunctionName=cisia_msfun  Parameters=Parameter1, Parameter2, Parameter3, resources, Parameter10, codeupdate, step_received, step_computed, dynamic_computed, step_sended, id_entity, id_project, id_type, name_type, color  mask(S-function:msfcn_unit_delay){Parameter1='SCADA_03', Parameter2=1, Parameter3='', resources=|, Parameter10=off, codeupdate=off, step_received=|, step_computed=, dynamic_computed=, step_sended=|, id_entity=510, id_project=6, id_type=125, name_type=SCADA, color=#FFFFFF}
      mask resources=|
      | *** INPUT RESOURCES ***
      | NUM_INPUTS 3
      | CYBER_FAULT (10)
      | POWER1 (1)
      | PLC_QoS (1)
      |
      | *** STATE VARIABLES ***
      | NUM_VARIABLES 14
      | Operative_Level(NUMERIC)(1)(1)
      | Dos_attack(NUMERIC)(1)(0)
      | MITM_attack(NUMERIC)(1)(0)
      | Virus_Attack(NUMERIC)(1)(0)
      | Port_Scan_Attack(NUMERIC)(1)(0)
      | Cyber_Fault(NUMERIC_ARRAY)(10)(0  0  0  0  0  0  0  0  0  0)
      | BGP_hijacking(NUMERIC)(1)(0)
      | Mechanical_Fault(NUMERIC)(1)(0)
      | BotNet_Attack(NUMERIC)(1)(0)
      | Data_Corruption(NUMERIC)(1)(0)
      | SW_Change(NUMERIC)(1)(0)
      | Config_Change(NUMERIC)(1)(0)
      | Port_Saturation(NUMERIC)(1)(0)
      | Control_Fault(NUMERIC)(1)(0)
      |
      | *** OUTPUT RESOURCES ***
      | NUM_OUTPUTS 2
      | CYBER_FAULT (10)
      | SCADA_QoS (1)
      mask step_received=|
      | Cyber_Fault=max(CYBER_FAULT, transpose([Dos_attack MITM_attack Virus_Attack Port_Scan_Attack  BGP_hijacking BotNet_Attack Data_Corruption SW_Change Config_Change Port_Saturation]));
      |
      |
      | %Control_Fault=max([Mechanical_Fault Dos_attack min(0.5,max(Cyber_Fault))]);
      |
      |
      |
      | %Operative_Level=min([1-max(Cyber_Fault) 1-Mechanical_Fault POWER1 PLC_QoS]);
      mask step_sended=|
      | SCADA_QoS=Operative_Level;
      |
      | CYBER_FAULT=Cyber_Fault.*transpose([0 0 0.5 0.2 0 0 0 0 0 0]);
      mask prompts: Parameter1 "entity name"; Parameter2 "sampling time"; Parameter3 "project"; resources "input resources and state variables"; Parameter10 "Bring state variables to output"; codeupdate "update code from mask"
      mask help: This is a level-2 MATLAB file S-function which demonstrates CISIA entity
      mask DialogControl Container1 Prompt: All parameters
      mask Display: image('Icons/SCADA.png');port_label('input',1,'\color{yellow}\spadesuit','texmode','on');port_label('input',2,'\color{yellow}\spadesuit','texmode','on')
  Second_Substation (518) : M-S-Function  FunctionName=cisia_msfun  Parameters=Parameter1, Parameter2, Parameter3, resources, Parameter10, codeupdate, step_received, step_computed, dynamic_computed, step_sended, id_entity, id_project, id_type, name_type, color  mask(S-function:msfcn_unit_delay){Parameter1='Second_Substation', Parameter2=1, Parameter3='SistemiIoT', resources=|, Parameter10=off, codeupdate=off, step_received=|, step_computed=, dynamic_computed=, step_sended=|, id_entity=518, id_project=6, id_type=94, name_type=PowerAvailability, color=#FFFFFF}
      mask resources=|
      | *** INPUT RESOURCES ***
      | NUM_INPUTS 1
      | POWER1 (1)
      |
      | *** STATE VARIABLES ***
      | NUM_VARIABLES 2
      | Operative_Level(NUMERIC)(1)(1)
      | Power_Fault(NUMERIC)(1)(0)
      |
      | *** OUTPUT RESOURCES ***
      | NUM_OUTPUTS 2
      | POWER1 (1)
      | POWER_QoS (1)
      mask step_received=|
      | Power_Fault=1-POWER1;
      | Operative_Level=1-Power_Fault;
      mask step_sended=|
      | POWER1=1-Power_Fault;
      | POWER_QoS=1-Power_Fault;
      mask prompts: Parameter1 "entity name"; Parameter2 "sampling time"; Parameter3 "project"; resources "input resources and state variables"; Parameter10 "Bring state variables to output"; codeupdate "update code from mask"
      mask help: This is a level-2 MATLAB file S-function which demonstrates CISIA entity
      mask DialogControl Container1 Prompt: All parameters
      mask Display: image('Icons/PowerAvailability.png')
  Tank_01 (334) : M-S-Function  FunctionName=cisia_msfun  Parameters=Parameter1, Parameter2, Parameter3, resources, Parameter10, codeupdate, step_received, step_computed, dynamic_computed, step_sended, id_entity, id_project, id_type, name_type, color  mask(S-function:msfcn_unit_delay){Parameter1='Tank_01', Parameter2=1, Parameter3='', resources=|, Parameter10=off, codeupdate=off, step_received=|, step_computed=Water_Level_new=max(0,Water_Level-0.2*Water_Fault);, dynamic_computed=, step_sended=WATER=Operative_Level;, id_entity=334, id_project=6, id_type=87, name_type=Water_Tank, color=#FFFFFF}
      mask resources=|
      | *** INPUT RESOURCES ***
      | NUM_INPUTS 1
      | WATER1 (1)
      |
      | *** STATE VARIABLES ***
      | NUM_VARIABLES 16
      | Operative_Level(NUMERIC)(1)(1)
      | Dos_attack(NUMERIC)(1)(0)
      | MITM_attack(NUMERIC)(1)(0)
      | Virus_Attack(NUMERIC)(1)(0)
      | Port_Scan_Attack(NUMERIC)(1)(0)
      | Cyber_Fault(NUMERIC_ARRAY)(10)(0  0  0  0  0  0  0  0  0  0)
      | BGP_hijacking(NUMERIC)(1)(0)
      | Mechanical_Fault(NUMERIC)(1)(0)
      | BotNet_Attack(NUMERIC)(1)(0)
      | Data_Corruption(NUMERIC)(1)(0)
      | SW_Change(NUMERIC)(1)(0)
      | Config_Change(NUMERIC)(1)(0)
      | Port_Saturation(NUMERIC)(1)(0)
      | Water_Fault(NUMERIC)(1)(0)
      | Water_Level(NUMERIC)(1)(1)
      | IoT_Fault(NUMERIC)(1)(0)
      |
      | *** OUTPUT RESOURCES ***
      | NUM_OUTPUTS 1
      | WATER1 (1)
      mask step_received=|
      | Water_Fault=1-WATER1;
      |
      | Operative_Level=min([1-Mechanical_Fault 1-Water_Fault]);
      mask prompts: Parameter1 "entity name"; Parameter2 "sampling time"; Parameter3 "project"; resources "input resources and state variables"; Parameter10 "Bring state variables to output"; codeupdate "update code from mask"
      mask help: This is a level-2 MATLAB file S-function which demonstrates CISIA entity
      mask DialogControl Container1 Prompt: All parameters
      mask Display: disp('Water_Tank')
  Toilette_01 (499) : M-S-Function  FunctionName=cisia_msfun  Parameters=Parameter1, Parameter2, Parameter3, resources, Parameter10, codeupdate, step_received, step_computed, dynamic_computed, step_sended, id_entity, id_project, id_type, name_type, color  mask(S-function:msfcn_unit_delay){Parameter1='Toilette_01', Parameter2=1, Parameter3='', resources=|, Parameter10=off, codeupdate=off, step_received=|, step_computed=, dynamic_computed=, step_sended=TOILETTE_QoS=Operative_Level;, id_entity=499, id_project=6, id_type=121, name_type=Toilette, color=#FFFFFF}
      mask resources=|
      | *** INPUT RESOURCES ***
      | NUM_INPUTS 2
      | POWER1 (1)
      | WATER1 (1)
      |
      | *** STATE VARIABLES ***
      | NUM_VARIABLES 3
      | Operative_Level(NUMERIC)(1)(1)
      | Power_Fault(NUMERIC)(1)(0)
      | Water_Fault(NUMERIC)(1)(0)
      |
      | *** OUTPUT RESOURCES ***
      | NUM_OUTPUTS 1
      | TOILETTE_QoS (1)
      mask step_received=|
      | Power_Fault=1-POWER;
      | Water_Fault=1-WATER;
      |
      | Operative_Level=min(1-Power_Fault,1-Water_Fault);
      mask prompts: Parameter1 "entity name"; Parameter2 "sampling time"; Parameter3 "project"; resources "input resources and state variables"; Parameter10 "Bring state variables to output"; codeupdate "update code from mask"
      mask help: This is a level-2 MATLAB file S-function which demonstrates CISIA entity
      mask DialogControl Container1 Prompt: All parameters
      mask Display: disp('Toilette');port_label('input',1,'\color{yellow}\spadesuit','texmode','on');port_label('input',2,'\color{yellow}\spadesuit','texmode','on')
  Valve_01 (511) : M-S-Function  FunctionName=cisia_msfun  Parameters=Parameter1, Parameter2, Parameter3, resources, Parameter10, codeupdate, step_received, step_computed, dynamic_computed, step_sended, id_entity, id_project, id_type, name_type, color  mask(S-function:msfcn_unit_delay){Parameter1='Valve_01', Parameter2=1, Parameter3='', resources=|, Parameter10=off, codeupdate=off, step_received=|, step_computed=, dynamic_computed=, step_sended=|, id_entity=511, id_project=6, id_type=126, name_type=Valve, color=#FFFFFF}
      mask resources=|
      | *** INPUT RESOURCES ***
      | NUM_INPUTS 3
      | CYBER_FAULT (10)
      | POWER1 (1)
      | TELECONTROL (1)
      |
      | *** STATE VARIABLES ***
      | NUM_VARIABLES 16
      | Operative_Level(NUMERIC)(1)(1)
      | Dos_attack(NUMERIC)(1)(0)
      | MITM_attack(NUMERIC)(1)(0)
      | Virus_Attack(NUMERIC)(1)(0)
      | Port_Scan_Attack(NUMERIC)(1)(0)
      | Cyber_Fault(NUMERIC_ARRAY)(10)(0  0  0  0  0  0  0  0  0  0)
      | BGP_hijacking(NUMERIC)(1)(0)
      | Mechanical_Fault(NUMERIC)(1)(0)
      | Unauthorized_Access(NUMERIC)(1)(0)
      | BotNet_Attack(NUMERIC)(1)(0)
      | Data_Corruption(NUMERIC)(1)(0)
      | Rouge_Access(NUMERIC)(1)(0)
      | SW_Change(NUMERIC)(1)(0)
      | Config_Change(NUMERIC)(1)(0)
      | Port_Saturation(NUMERIC)(1)(0)
      | Control_Fault(NUMERIC)(1)(0)
      |
      | *** OUTPUT RESOURCES ***
      | NUM_OUTPUTS 2
      | CYBER_FAULT (10)
      | VALVE_QoS (1)
      mask step_received=|
      | Cyber_Fault=max(CYBER_FAULT, transpose([Dos_attack MITM_attack Virus_Attack Port_Scan_Attack  BGP_hijacking BotNet_Attack Data_Corruption SW_Change Config_Change Port_Saturation]));
      |
      |
      | Control_Fault=max([1-TELECONTROL Mechanical_Fault Dos_attack min(0.5,max(Cyber_Fault))]);
      |
      |
      |
      | Operative_Level=min([1-max(Cyber_Fault) 1-Mechanical_Fault POWER]);
      mask step_sended=|
      | VALVE_QoS=Operative_Level;
      |
      | CYBER_FAULT=Cyber_Fault.*transpose([0 0 0.5 0.2 0 0 0 0 0 0]);
      mask prompts: Parameter1 "entity name"; Parameter2 "sampling time"; Parameter3 "project"; resources "input resources and state variables"; Parameter10 "Bring state variables to output"; codeupdate "update code from mask"
      mask help: This is a level-2 MATLAB file S-function which demonstrates CISIA entity
      mask DialogControl Container1 Prompt: All parameters
      mask Display: image('Icons/Valve.png');port_label('input',1,'\color{yellow}\spadesuit','texmode','on');port_label('input',2,'\color{yellow}\spadesuit','texmode','on')
  Valve_02 (512) : M-S-Function  FunctionName=cisia_msfun  Parameters=Parameter1, Parameter2, Parameter3, resources, Parameter10, codeupdate, step_received, step_computed, dynamic_computed, step_sended, id_entity, id_project, id_type, name_type, color  mask(S-function:msfcn_unit_delay){Parameter1='Valve_02', Parameter2=1, Parameter3='', resources=|, Parameter10=off, codeupdate=off, step_received=|, step_computed=, dynamic_computed=, step_sended=|, id_entity=512, id_project=6, id_type=126, name_type=Valve, color=#FFFFFF}
      mask resources=|
      | *** INPUT RESOURCES ***
      | NUM_INPUTS 3
      | CYBER_FAULT (10)
      | POWER1 (1)
      | TELECONTROL (1)
      |
      | *** STATE VARIABLES ***
      | NUM_VARIABLES 16
      | Operative_Level(NUMERIC)(1)(1)
      | Dos_attack(NUMERIC)(1)(0)
      | MITM_attack(NUMERIC)(1)(0)
      | Virus_Attack(NUMERIC)(1)(0)
      | Port_Scan_Attack(NUMERIC)(1)(0)
      | Cyber_Fault(NUMERIC_ARRAY)(10)(0  0  0  0  0  0  0  0  0  0)
      | BGP_hijacking(NUMERIC)(1)(0)
      | Mechanical_Fault(NUMERIC)(1)(0)
      | Unauthorized_Access(NUMERIC)(1)(0)
      | BotNet_Attack(NUMERIC)(1)(0)
      | Data_Corruption(NUMERIC)(1)(0)
      | Rouge_Access(NUMERIC)(1)(0)
      | SW_Change(NUMERIC)(1)(0)
      | Config_Change(NUMERIC)(1)(0)
      | Port_Saturation(NUMERIC)(1)(0)
      | Control_Fault(NUMERIC)(1)(0)
      |
      | *** OUTPUT RESOURCES ***
      | NUM_OUTPUTS 2
      | CYBER_FAULT (10)
      | VALVE_QoS (1)
      mask step_received=|
      | Cyber_Fault=max(CYBER_FAULT, transpose([Dos_attack MITM_attack Virus_Attack Port_Scan_Attack  BGP_hijacking BotNet_Attack Data_Corruption SW_Change Config_Change Port_Saturation]));
      |
      |
      | Control_Fault=max([1-TELECONTROL Mechanical_Fault Dos_attack min(0.5,max(Cyber_Fault))]);
      |
      |
      |
      | Operative_Level=min([1-max(Cyber_Fault) 1-Mechanical_Fault POWER]);
      mask step_sended=|
      | VALVE_QoS=Operative_Level;
      |
      | CYBER_FAULT=Cyber_Fault.*transpose([0 0 0.5 0.2 0 0 0 0 0 0]);
      mask prompts: Parameter1 "entity name"; Parameter2 "sampling time"; Parameter3 "project"; resources "input resources and state variables"; Parameter10 "Bring state variables to output"; codeupdate "update code from mask"
      mask help: This is a level-2 MATLAB file S-function which demonstrates CISIA entity
      mask DialogControl Container1 Prompt: All parameters
      mask Display: image('Icons/Valve.png');port_label('input',1,'\color{yellow}\spadesuit','texmode','on');port_label('input',2,'\color{yellow}\spadesuit','texmode','on')
  Valve_03 (513) : M-S-Function  FunctionName=cisia_msfun  Parameters=Parameter1, Parameter2, Parameter3, resources, Parameter10, codeupdate, step_received, step_computed, dynamic_computed, step_sended, id_entity, id_project, id_type, name_type, color  mask(S-function:msfcn_unit_delay){Parameter1='Valve_03', Parameter2=1, Parameter3='', resources=|, Parameter10=off, codeupdate=off, step_received=|, step_computed=, dynamic_computed=, step_sended=|, id_entity=513, id_project=6, id_type=126, name_type=Valve, color=#FFFFFF}
      mask resources=|
      | *** INPUT RESOURCES ***
      | NUM_INPUTS 3
      | CYBER_FAULT (10)
      | POWER1 (1)
      | TELECONTROL (1)
      |
      | *** STATE VARIABLES ***
      | NUM_VARIABLES 16
      | Operative_Level(NUMERIC)(1)(1)
      | Dos_attack(NUMERIC)(1)(0)
      | MITM_attack(NUMERIC)(1)(0)
      | Virus_Attack(NUMERIC)(1)(0)
      | Port_Scan_Attack(NUMERIC)(1)(0)
      | Cyber_Fault(NUMERIC_ARRAY)(10)(0  0  0  0  0  0  0  0  0  0)
      | BGP_hijacking(NUMERIC)(1)(0)
      | Mechanical_Fault(NUMERIC)(1)(0)
      | Unauthorized_Access(NUMERIC)(1)(0)
      | BotNet_Attack(NUMERIC)(1)(0)
      | Data_Corruption(NUMERIC)(1)(0)
      | Rouge_Access(NUMERIC)(1)(0)
      | SW_Change(NUMERIC)(1)(0)
      | Config_Change(NUMERIC)(1)(0)
      | Port_Saturation(NUMERIC)(1)(0)
      | Control_Fault(NUMERIC)(1)(0)
      |
      | *** OUTPUT RESOURCES ***
      | NUM_OUTPUTS 2
      | CYBER_FAULT (10)
      | VALVE_QoS (1)
      mask step_received=|
      | Cyber_Fault=max(CYBER_FAULT, transpose([Dos_attack MITM_attack Virus_Attack Port_Scan_Attack  BGP_hijacking BotNet_Attack Data_Corruption SW_Change Config_Change Port_Saturation]));
      |
      |
      | Control_Fault=max([1-TELECONTROL Mechanical_Fault Dos_attack min(0.5,max(Cyber_Fault))]);
      |
      |
      |
      | Operative_Level=min([1-max(Cyber_Fault) 1-Mechanical_Fault POWER]);
      mask step_sended=|
      | VALVE_QoS=Operative_Level;
      |
      | CYBER_FAULT=Cyber_Fault.*transpose([0 0 0.5 0.2 0 0 0 0 0 0]);
      mask prompts: Parameter1 "entity name"; Parameter2 "sampling time"; Parameter3 "project"; resources "input resources and state variables"; Parameter10 "Bring state variables to output"; codeupdate "update code from mask"
      mask help: This is a level-2 MATLAB file S-function which demonstrates CISIA entity
      mask DialogControl Container1 Prompt: All parameters
      mask Display: image('Icons/Valve.png');port_label('input',1,'\color{yellow}\spadesuit','texmode','on');port_label('input',2,'\color{yellow}\spadesuit','texmode','on')
  Valve_04 (514) : M-S-Function  FunctionName=cisia_msfun  Parameters=Parameter1, Parameter2, Parameter3, resources, Parameter10, codeupdate, step_received, step_computed, dynamic_computed, step_sended, id_entity, id_project, id_type, name_type, color  mask(S-function:msfcn_unit_delay){Parameter1='Valve_04', Parameter2=1, Parameter3='', resources=|, Parameter10=off, codeupdate=off, step_received=|, step_computed=, dynamic_computed=, step_sended=|, id_entity=514, id_project=6, id_type=126, name_type=Valve, color=#FFFFFF}
      mask resources=|
      | *** INPUT RESOURCES ***
      | NUM_INPUTS 3
      | CYBER_FAULT (10)
      | POWER1 (1)
      | TELECONTROL (1)
      |
      | *** STATE VARIABLES ***
      | NUM_VARIABLES 16
      | Operative_Level(NUMERIC)(1)(1)
      | Dos_attack(NUMERIC)(1)(0)
      | MITM_attack(NUMERIC)(1)(0)
      | Virus_Attack(NUMERIC)(1)(0)
      | Port_Scan_Attack(NUMERIC)(1)(0)
      | Cyber_Fault(NUMERIC_ARRAY)(10)(0  0  0  0  0  0  0  0  0  0)
      | BGP_hijacking(NUMERIC)(1)(0)
      | Mechanical_Fault(NUMERIC)(1)(0)
      | Unauthorized_Access(NUMERIC)(1)(0)
      | BotNet_Attack(NUMERIC)(1)(0)
      | Data_Corruption(NUMERIC)(1)(0)
      | Rouge_Access(NUMERIC)(1)(0)
      | SW_Change(NUMERIC)(1)(0)
      | Config_Change(NUMERIC)(1)(0)
      | Port_Saturation(NUMERIC)(1)(0)
      | Control_Fault(NUMERIC)(1)(0)
      |
      | *** OUTPUT RESOURCES ***
      | NUM_OUTPUTS 2
      | CYBER_FAULT (10)
      | VALVE_QoS (1)
      mask step_received=|
      | Cyber_Fault=max(CYBER_FAULT, transpose([Dos_attack MITM_attack Virus_Attack Port_Scan_Attack  BGP_hijacking BotNet_Attack Data_Corruption SW_Change Config_Change Port_Saturation]));
      |
      |
      | Control_Fault=max([1-TELECONTROL Mechanical_Fault Dos_attack min(0.5,max(Cyber_Fault))]);
      |
      |
      |
      | Operative_Level=min([1-max(Cyber_Fault) 1-Mechanical_Fault POWER]);
      mask step_sended=|
      | VALVE_QoS=Operative_Level;
      |
      | CYBER_FAULT=Cyber_Fault.*transpose([0 0 0.5 0.2 0 0 0 0 0 0]);
      mask prompts: Parameter1 "entity name"; Parameter2 "sampling time"; Parameter3 "project"; resources "input resources and state variables"; Parameter10 "Bring state variables to output"; codeupdate "update code from mask"
      mask help: This is a level-2 MATLAB file S-function which demonstrates CISIA entity
      mask DialogControl Container1 Prompt: All parameters
      mask Display: image('Icons/Valve.png');port_label('input',1,'\color{yellow}\spadesuit','texmode','on');port_label('input',2,'\color{yellow}\spadesuit','texmode','on')
  Valve_05 (515) : M-S-Function  FunctionName=cisia_msfun  Parameters=Parameter1, Parameter2, Parameter3, resources, Parameter10, codeupdate, step_received, step_computed, dynamic_computed, step_sended, id_entity, id_project, id_type, name_type, color  mask(S-function:msfcn_unit_delay){Parameter1='Valve_05', Parameter2=1, Parameter3='', resources=|, Parameter10=off, codeupdate=off, step_received=|, step_computed=, dynamic_computed=, step_sended=|, id_entity=515, id_project=6, id_type=126, name_type=Valve, color=#FFFFFF}
      mask resources=|
      | *** INPUT RESOURCES ***
      | NUM_INPUTS 3
      | CYBER_FAULT (10)
      | POWER1 (1)
      | TELECONTROL (1)
      |
      | *** STATE VARIABLES ***
      | NUM_VARIABLES 16
      | Operative_Level(NUMERIC)(1)(1)
      | Dos_attack(NUMERIC)(1)(0)
      | MITM_attack(NUMERIC)(1)(0)
      | Virus_Attack(NUMERIC)(1)(0)
      | Port_Scan_Attack(NUMERIC)(1)(0)
      | Cyber_Fault(NUMERIC_ARRAY)(10)(0  0  0  0  0  0  0  0  0  0)
      | BGP_hijacking(NUMERIC)(1)(0)
      | Mechanical_Fault(NUMERIC)(1)(0)
      | Unauthorized_Access(NUMERIC)(1)(0)
      | BotNet_Attack(NUMERIC)(1)(0)
      | Data_Corruption(NUMERIC)(1)(0)
      | Rouge_Access(NUMERIC)(1)(0)
      | SW_Change(NUMERIC)(1)(0)
      | Config_Change(NUMERIC)(1)(0)
      | Port_Saturation(NUMERIC)(1)(0)
      | Control_Fault(NUMERIC)(1)(0)
      |
      | *** OUTPUT RESOURCES ***
      | NUM_OUTPUTS 2
      | CYBER_FAULT (10)
      | VALVE_QoS (1)
      mask step_received=|
      | Cyber_Fault=max(CYBER_FAULT, transpose([Dos_attack MITM_attack Virus_Attack Port_Scan_Attack  BGP_hijacking BotNet_Attack Data_Corruption SW_Change Config_Change Port_Saturation]));
      |
      |
      | Control_Fault=max([1-TELECONTROL Mechanical_Fault Dos_attack min(0.5,max(Cyber_Fault))]);
      |
      |
      |
      | Operative_Level=min([1-max(Cyber_Fault) 1-Mechanical_Fault POWER]);
      mask step_sended=|
      | VALVE_QoS=Operative_Level;
      |
      | CYBER_FAULT=Cyber_Fault.*transpose([0 0 0.5 0.2 0 0 0 0 0 0]);
      mask prompts: Parameter1 "entity name"; Parameter2 "sampling time"; Parameter3 "project"; resources "input resources and state variables"; Parameter10 "Bring state variables to output"; codeupdate "update code from mask"
      mask help: This is a level-2 MATLAB file S-function which demonstrates CISIA entity
      mask DialogControl Container1 Prompt: All parameters
      mask Display: image('Icons/Valve.png');port_label('input',1,'\color{yellow}\spadesuit','texmode','on');port_label('input',2,'\color{yellow}\spadesuit','texmode','on')
  Water_Availability (516) : M-S-Function  FunctionName=cisia_msfun  Parameters=Parameter1, Parameter2, Parameter3, resources, Parameter10, codeupdate, step_received, step_computed, dynamic_computed, step_sended, id_entity, id_project, id_type, name_type, color  mask(S-function:msfcn_unit_delay){Parameter1='Water_Availability', Parameter2=1, Parameter3='', resources=|, Parameter10=off, codeupdate=off, step_received=|, step_computed=, dynamic_computed=, step_sended=|, id_entity=516, id_project=6, id_type=127, name_type=Water_Availability, color=#FFFFFF}
      mask resources=|
      | *** INPUT RESOURCES ***
      | NUM_INPUTS 1
      | WATER1 (1)
      |
      | *** STATE VARIABLES ***
      | NUM_VARIABLES 2
      | Operative_Level(NUMERIC)(1)(1)
      | Water_Fault(NUMERIC)(1)(0)
      |
      | *** OUTPUT RESOURCES ***
      | NUM_OUTPUTS 2
      | WATER1 (1)
      | WATER_QoS (1)
      mask step_received=|
      | Water_Fault=1-WATER;
      |
      | Operative_Level=1-Water_Fault;
      mask step_sended=|
      | WATER=1-Water_Fault;
      | WATER_QoS = 1-Water_Fault;
      mask prompts: Parameter1 "entity name"; Parameter2 "sampling time"; Parameter3 "project"; resources "input resources and state variables"; Parameter10 "Bring state variables to output"; codeupdate "update code from mask"
      mask help: This is a level-2 MATLAB file S-function which demonstrates CISIA entity
      mask DialogControl Container1 Prompt: All parameters
      mask Display: image('Icons/Water_Availability.png');port_label('input',1,'\color{yellow}\spadesuit','texmode','on')
  Water_pipe_01 (505) : M-S-Function  FunctionName=cisia_msfun  Parameters=Parameter1, Parameter2, Parameter3, resources, Parameter10, codeupdate, step_received, step_computed, dynamic_computed, step_sended, id_entity, id_project, id_type, name_type, color  mask(S-function:msfcn_unit_delay){Parameter1='Water_pipe_01', Parameter2=1, Parameter3='', resources=|, Parameter10=off, codeupdate=off, step_received=|, step_computed=, dynamic_computed=, step_sended=WATER=1-Water_Fault;, id_entity=505, id_project=6, id_type=122, name_type=Water_Pipe, color=#00FFFF}
      mask resources=|
      | *** INPUT RESOURCES ***
      | NUM_INPUTS 2
      | WATER1 (1)
      | VALVE_QoS (1)
      |
      | *** STATE VARIABLES ***
      | NUM_VARIABLES 3
      | Operative_Level(NUMERIC)(1)(1)
      | Mechanical_Fault(NUMERIC)(1)(0)
      | Water_Fault(NUMERIC)(1)(0)
      |
      | *** OUTPUT RESOURCES ***
      | NUM_OUTPUTS 1
      | WATER1 (1)
      mask step_received=|
      | Water_Fault=max([1-WATER1 Mechanical_Fault 1-VALVE_QoS]);
      |
      | Operative_Level=1-Water_Fault;
      mask prompts: Parameter1 "entity name"; Parameter2 "sampling time"; Parameter3 "project"; resources "input resources and state variables"; Parameter10 "Bring state variables to output"; codeupdate "update code from mask"
      mask help: This is a level-2 MATLAB file S-function which demonstrates CISIA entity
      mask DialogControl Container1 Prompt: All parameters
      mask Display: disp('Water_Pipe');port_label('input',2,'\color{yellow}\spadesuit','texmode','on')
  Water_pipe_02 (503) : M-S-Function  FunctionName=cisia_msfun  Parameters=Parameter1, Parameter2, Parameter3, resources, Parameter10, codeupdate, step_received, step_computed, dynamic_computed, step_sended, id_entity, id_project, id_type, name_type, color  mask(S-function:msfcn_unit_delay){Parameter1='Water_pipe_02', Parameter2=1, Parameter3='', resources=|, Parameter10=off, codeupdate=off, step_received=|, step_computed=, dynamic_computed=, step_sended=WATER=1-Water_Fault;, id_entity=503, id_project=6, id_type=122, name_type=Water_Pipe, color=#00FFFF}
      mask resources=|
      | *** INPUT RESOURCES ***
      | NUM_INPUTS 2
      | WATER1 (1)
      | VALVE_QoS (1)
      |
      | *** STATE VARIABLES ***
      | NUM_VARIABLES 3
      | Operative_Level(NUMERIC)(1)(1)
      | Mechanical_Fault(NUMERIC)(1)(0)
      | Water_Fault(NUMERIC)(1)(0)
      |
      | *** OUTPUT RESOURCES ***
      | NUM_OUTPUTS 1
      | WATER1 (1)
      mask step_received=|
      | Water_Fault=max([1-WATER1 Mechanical_Fault 1-VALVE_QoS]);
      |
      | Operative_Level=1-Water_Fault;
      mask prompts: Parameter1 "entity name"; Parameter2 "sampling time"; Parameter3 "project"; resources "input resources and state variables"; Parameter10 "Bring state variables to output"; codeupdate "update code from mask"
      mask help: This is a level-2 MATLAB file S-function which demonstrates CISIA entity
      mask DialogControl Container1 Prompt: All parameters
      mask Display: disp('Water_Pipe');port_label('input',2,'\color{yellow}\spadesuit','texmode','on')
  Water_pipe_03 (504) : M-S-Function  FunctionName=cisia_msfun  Parameters=Parameter1, Parameter2, Parameter3, resources, Parameter10, codeupdate, step_received, step_computed, dynamic_computed, step_sended, id_entity, id_project, id_type, name_type, color  mask(S-function:msfcn_unit_delay){Parameter1='Water_pipe_03', Parameter2=1, Parameter3='', resources=|, Parameter10=off, codeupdate=off, step_received=|, step_computed=, dynamic_computed=, step_sended=WATER=1-Water_Fault;, id_entity=504, id_project=6, id_type=122, name_type=Water_Pipe, color=#00FFFF}
      mask resources=|
      | *** INPUT RESOURCES ***
      | NUM_INPUTS 2
      | WATER1 (1)
      | VALVE_QoS (1)
      |
      | *** STATE VARIABLES ***
      | NUM_VARIABLES 3
      | Operative_Level(NUMERIC)(1)(1)
      | Mechanical_Fault(NUMERIC)(1)(0)
      | Water_Fault(NUMERIC)(1)(0)
      |
      | *** OUTPUT RESOURCES ***
      | NUM_OUTPUTS 1
      | WATER1 (1)
      mask step_received=|
      | Water_Fault=max([1-WATER1 Mechanical_Fault 1-VALVE_QoS]);
      |
      | Operative_Level=1-Water_Fault;
      mask prompts: Parameter1 "entity name"; Parameter2 "sampling time"; Parameter3 "project"; resources "input resources and state variables"; Parameter10 "Bring state variables to output"; codeupdate "update code from mask"
      mask help: This is a level-2 MATLAB file S-function which demonstrates CISIA entity
      mask DialogControl Container1 Prompt: All parameters
      mask Display: disp('Water_Pipe');port_label('input',2,'\color{yellow}\spadesuit','texmode','on')
  media : MATLAB Function  TreatAsAtomicUnit=on
  media1 : MATLAB Function  TreatAsAtomicUnit=on
  media2 : MATLAB Function  TreatAsAtomicUnit=on
  media3 : MATLAB Function  TreatAsAtomicUnit=on
  media4 : MATLAB Function  TreatAsAtomicUnit=on
  wires:
  media/1(y) -> [SCADA_QoS], SAVE_SCADA (26)/1  "SCADA_QoS"
  CISIA_MASTER (0)/1 -> Display18/1  "MINOR HITS"
  CISIA_MASTER (0)/2 -> Display19/1  "MAJOR HITS"
  CISIA_MASTER (0)/4 -> Display21/1  "TIME PAST"
  CISIA_MASTER (0)/3 -> Display20/1  "DELTA TIME"
  Mux/1 -> media/1(u)
  Mux1/1 -> media1/1(u)
  media1/1(y) -> [PLC_QoS], SAVE_PLC (31)/1  "PLC_QoS"
  [VALVE_QoS_03] -> Water_pipe_01 (505)/2
  Valve_03 (513)/2 -> [VALVE_QoS_03]  "VALVE_QoS"
  Valve_04 (514)/2 -> [VALVE_QoS_04]  "VALVE_QoS"
  [VALVE_QoS_04] -> Water_pipe_02 (503)/2
  [VALVE_QoS_05] -> Water_pipe_03 (504)/2
  Valve_05 (515)/2 -> [VALVE_QoS_05]  "VALVE_QoS"
  Valve_03 (513)/1 -> [Cyber_Fault_V03]  "CYBER_FAULT"
  Valve_04 (514)/1 -> [Cyber_Fault_V04]  "CYBER_FAULT"
  [Cyber_Fault_V03] -> MinMax/1
  [Cyber_Fault_V04] -> MinMax/2
  Valve_05 (515)/1 -> [Cyber_Fault_V05]  "CYBER_FAULT"
  [Cyber_Fault_V05] -> MinMax/3
  SCADA_03 (510)/1 -> [Cyber_Fault_S3]  "CYBER_FAULT"
  Tank_01 (334)/1 -> Water_pipe_03 (504)/1, Water_pipe_02 (503)/1, Water_pipe_01 (505)/1  "WATER1"
  [Cyber_Fault_S3] -> MinMax/4
  [Cyber_Fault_PLC3] -> Valve_03 (513)/1
  SCADA_03 (510)/2 -> [SCADA3_QoS]  "SCADA_QoS"
  [Cyber_Fault_PLC3] -> SCADA_03 (510)/1
  PLC_03 (507)/3 -> SCADA_03 (510)/3, [PLC3_QoS]  "PLC_QoS"
  PLC_03 (507)/1 -> [Cyber_Fault_PLC3]  "CYBER_FAULT"
  PLC_03 (507)/2 -> Valve_05 (515)/3, Valve_04 (514)/3, Valve_03 (513)/3  "TELECONTROL"
  MinMax/1 -> PLC_03 (507)/1
  Market_01 (517)/1 -> [MARKET_QoS]  "MARKET_QoS"
  Pump_01 (502)/1 -> [PUMP_QoS]  "PUMP_QoS"
  PLC_01 (501)/1 -> Generator_01 (495)/1, [Cyber_Fault_PLC1]  "CYBER_FAULT"
  [Cyber_Fault_PLC1] -> SCADA_01 (508)/1
  PLC_01 (501)/3 -> SCADA_01 (508)/3, [PLC1_QoS]  "PLC_QoS"
  Constant2/1 -> Second_Substation (518)/1  "POWER1"
  MinMax17/1 -> [Power_esterno]
  [Power_esterno] -> PowerTower_01 (497)/1
  [Cyber_Fault_PLC3] -> Valve_04 (514)/1
  [Cyber_Fault_PLC3] -> Valve_05 (515)/1
  [Power_esterno] -> MinMax3/2
  [Power_interno] -> MinMax3/1
  MinMax3/1 -> SCADA_01 (508)/2
  [Cyber_Fault_PLC2] -> SCADA_02 (509)/1
  PLC_02 (506)/3 -> [PLC2_QoS], SCADA_02 (509)/3  "PLC_QoS"
  SCADA_02 (509)/2 -> [SCADA2_QoS]  "SCADA_QoS"
  SCADA_02 (509)/1 -> [Cyber_Fault_S2]  "CYBER_FAULT"
  MinMax1/1 -> PLC_02 (506)/1
  PLC_02 (506)/1 -> [Cyber_Fault_PLC2]  "CYBER_FAULT"
  [Cyber_Fault_S2] -> MinMax1/3
  [Cyber_Fault_PLC2] -> Valve_01 (511)/1
  [Cyber_Fault_PLC2] -> Valve_02 (512)/1
  PLC_02 (506)/2 -> Valve_02 (512)/3, Valve_01 (511)/3  "TELECONTROL"
  [Cyber_Fault_V02] -> MinMax1/2
  [Cyber_Fault_V01] -> MinMax1/1
  Fuel_Tank_01 (494)/1 -> Fuel_pipe_02 (493)/2, Fuel_pipe_01 (492)/2  "FUEL"
  [VALVE_QoS_01] -> Fuel_pipe_01 (492)/1
  [VALVE_QoS_02] -> Fuel_pipe_02 (493)/1
  Fuel_pipe_02 (493)/1 -> [Fuel_2]  "FUEL"
  Power_availability (362)/2 -> [POWER1_QoS]  "POWER_QoS"
  Second_Substation (518)/2 -> [POWER2_QoS]  "POWER_QoS"
  Power_availability (362)/1 -> MinMax17/1  "POWER1"
  Second_Substation (518)/1 -> MinMax17/2  "POWER1"
  PowerTower_01 (497)/1 -> [TOWER_QoS]  "TOWER_QoS"
  Water_pipe_01 (505)/1 -> [Water_1]  "WATER1"
  [Water_1] -> Market_01 (517)/2
  Water_pipe_02 (503)/1 -> [Water_2]  "WATER1"
  [Water_2] -> Toilette_01 (499)/2
  Water_pipe_03 (504)/1 -> [Water_3]  "WATER1"
  Fuel_pipe_01 (492)/1 -> [Fuel_1]  "FUEL"
  [Fuel_1] -> Pump_01 (502)/2
  Water_Availability (516)/2 -> [WATER_QoS]  "WATER_QoS"
  [SCADA1_QoS] -> Mux/1
  [SCADA2_QoS] -> Mux/2
  [SCADA3_QoS] -> Mux/3
  [PLC1_QoS] -> Mux1/1
  [PLC2_QoS] -> Mux1/2
  [PLC3_QoS] -> Mux1/3
  [WATER_QoS] -> SAVE_WATER (32)/1  "WATER_QoS"
  media2/1(y) -> [POWER_QoS], SAVE_17 (17)/1  "POWER_QoS"
  Mux2/1 -> media2/1(u)
  [POWER1_QoS] -> Mux2/1
  [POWER2_QoS] -> Mux2/2
  [GENERATOR_QoS] -> Mux2/3
  media3/1(y) -> SAVE_VALVE (25)/1  "VALVE_QoS"
  Mux4/1 -> media3/1(u)
  Fuel_Tank_01 (494)/2 -> [FUEL_QoS]  "FUEL_QoS"
  [FUEL_QoS] -> SAVE_FUEL (34)/1  "FUEL_QoS"
  media4/1(y) -> SAVE_GENERAL (33)/1  "GENERAL_QoS"
  Mux6/1 -> media4/1(u)
  [VALVE_QoS_01] -> Mux4/1
  [VALVE_QoS_02] -> Mux4/2
  [VALVE_QoS_03] -> Mux4/3
  [VALVE_QoS_04] -> Mux4/4
  [VALVE_QoS_05] -> Mux4/5
  [MARKET_QoS] -> SAVE_MARKET (28)/1  "MARKET_QoS"
  [TOILETTE_QoS] -> SAVE_TOILETTE (27)/1  "WC_QoS"
  [CARWASH_QoS] -> SAVE_CAR (29)/1  "CW_QoS"
  [TOWER_QoS] -> SAVE_TOWER (35)/1  "TOWER_QoS"
  [PUMP_QoS] -> SAVE_PUMP (30)/1  "PUMP_QoS"
  [SCADA_QoS] -> Mux6/1
  [PLC_QoS] -> Mux6/2
  [POWER_QoS] -> Mux6/3
  [WATER_QoS] -> Mux6/4
  [FUEL_QoS] -> Mux6/5
  Toilette_01 (499)/1 -> [TOILETTE_QoS]  "TOILETTE_QoS"
  [Fuel_2] -> Generator_01 (495)/3
  PLC_01 (501)/2 -> Generator_01 (495)/2  "TELECONTROL"
  MinMax2/1 -> PLC_01 (501)/1
  [Cyber_Fault_S1] -> MinMax2/2
  [Cyber_Fault_GEN] -> MinMax2/1
  Water_Availability (516)/1 -> Tank_01 (334)/1  "WATER1"
  Valve_01 (511)/1 -> [Cyber_Fault_V01]  "CYBER_FAULT"
  Valve_01 (511)/2 -> [VALVE_QoS_01]  "VALVE_QoS"
  Valve_02 (512)/2 -> [VALVE_QoS_02]  "VALVE_QoS"
  Valve_02 (512)/1 -> [Cyber_Fault_V02]  "CYBER_FAULT"
  SCADA_01 (508)/2 -> [SCADA1_QoS]  "SCADA_QoS"
  SCADA_01 (508)/1 -> [Cyber_Fault_S1]  "CYBER_FAULT"
  Generator_01 (495)/1 -> [Cyber_Fault_GEN]  "CYBER_FAULT"
  Generator_01 (495)/2 -> [Power_interno]  "POWER1"
  Generator_01 (495)/3 -> [GENERATOR_QoS]  "GENERATOR_QoS"
  [Power_interno] -> MinMax4/1
  [Power_esterno] -> MinMax4/2
  MinMax4/1 -> PLC_01 (501)/2
  [Power_interno] -> MinMax5/1
  [Power_esterno] -> MinMax5/2
  MinMax5/1 -> SCADA_02 (509)/2
  [Power_interno] -> MinMax6/1
  [Power_esterno] -> MinMax6/2
  MinMax6/1 -> PLC_02 (506)/2
  [Power_interno] -> MinMax7/1
  [Power_esterno] -> MinMax7/2
  MinMax7/1 -> Valve_01 (511)/2
  [Power_interno] -> MinMax8/1
  [Power_esterno] -> MinMax8/2
  MinMax8/1 -> Valve_02 (512)/2
  [Power_interno] -> MinMax9/1
  [Power_esterno] -> MinMax9/2
  MinMax9/1 -> PLC_03 (507)/2
  [Power_interno] -> MinMax10/1
  [Power_esterno] -> MinMax10/2
  MinMax10/1 -> SCADA_03 (510)/2
  [Power_interno] -> MinMax11/1
  [Power_esterno] -> MinMax11/2
  MinMax11/1 -> Valve_03 (513)/2
  [Power_interno] -> MinMax12/1
  [Power_esterno] -> MinMax12/2
  MinMax12/1 -> Valve_04 (514)/2
  [Power_interno] -> MinMax13/1
  [Power_esterno] -> MinMax13/2
  MinMax13/1 -> Valve_05 (515)/2
  [Power_interno] -> MinMax14/1
  [Power_esterno] -> MinMax14/2
  MinMax14/1 -> Market_01 (517)/1
  [Power_interno] -> MinMax15/1
  [Power_esterno] -> MinMax15/2
  MinMax15/1 -> Toilette_01 (499)/1
  [Power_interno] -> MinMax16/1
  [Power_esterno] -> MinMax16/2
  MinMax16/1 -> Pump_01 (502)/1
  CarWash_01 (491)/1 -> [CARWASH_QoS]  "CARWASH_QoS"
  [Power_esterno] -> CarWash_01 (491)/1
  [Water_3] -> CarWash_01 (491)/2
